simulink model "aurora_cpu_ch0_ver2_rtxsg"  (R2019b)
(part 3 of 4)

\"ch19\":{\"PauseBehavior\":\"0\",\"IdleBehavior\":\"0\",\"DefaultValueReg\":\"0\"},\"ch20\":{\"PauseBehavior\":\"0\",\"IdleBehavior\":\"0\",\"DefaultValueReg\":\"0\"},\"ch21\":{\"PauseBehavior\":\"0\",\"IdleBehavior\":\"0\",\"DefaultValueReg\":\"0\"},\"ch22\":{\"PauseBehavior\":\"0\",\"IdleBehavior\":\"0\",\"DefaultValueReg\":\"0\"},\"ch23\":{\"PauseBehavior\":\"0\",\"IdleBehavior\":\"0\",\"DefaultValueReg\":\"0\"},\"ch24\":{\"PauseBehavior\":\"0\",\"IdleBehavior\":\"0\",\"DefaultValueReg\":\"0\"},\"ch25\":{\"PauseBehavior\":\"0\",\"IdleBehavior\":\"0\",\"DefaultValueReg\":\"0\"},\"ch26\":{\"PauseBehavior\":\"0\",\"IdleBehavior\":\"0\",\"DefaultValueReg\":\"0\"},\"ch27\":{\"PauseBehavior\":\"0\",\"IdleBehavior\":\"0\",\"DefaultValueReg\":\"0\"},\"ch28\":{\"PauseBehavior\":\"0\",\"IdleBehavior\":\"0\",\"DefaultValueReg\":\"0\"},\"ch29\":{\"PauseBehavior\":\"0\",\"IdleBehavior\":\"0\",\"DefaultValueReg\":\"0\"},\"ch30\":{\"PauseBehavior\":\"0\",\"IdleBehavior\":\"0\",\"DefaultValueReg\":\"0\"},\"ch31\":{\"PauseBehavior\":\"0\",\"IdleBehavior\":\"0\",\"DefaultValueReg\":\"0\"}}}"  Expansion_DV_4B="{\"dv_Expansion_4B\":{\"ch0\":{\"PauseBehavior\":\"0\",\"IdleBehavior\":\"0\",\"DefaultValueReg\":\"0\"},\"ch1\":{\"PauseBehavior\":\"0\",\"IdleBehavior\":\"0\",\"DefaultValueReg\":\"0\"},\"ch2\":{\"PauseBehavior\":\"0\",\"IdleBehavior\":\"0\",\"DefaultValueReg\":\"0\"},\"ch3\":{\"PauseBehavior\":\"0\",\"IdleBehavior\":\"0\",\"DefaultValueReg\":\"0\"},\"ch4\":{\"PauseBehavior\":\"0\",\"IdleBehavior\":\"0\",\"DefaultValueReg\":\"0\"},\"ch5\":{\"PauseBehavior\":\"0\",\"IdleBehavior\":\"0\",\"DefaultValueReg\":\"0\"},\"ch6\":{\"PauseBehavior\":\"0\",\"IdleBehavior\":\"0\",\"DefaultValueReg\":\"0\"},\"ch7\":{\"PauseBehavior\":\"0\",\"IdleBehavior\":\"0\",\"DefaultValueReg\":\"0\"},\"ch8\":{\"PauseBehavior\":\"0\",\"IdleBehavior\":\"0\",\"DefaultValueReg\":\"0\"},\"ch9\":{\"PauseBehavior\":\"0\",\"IdleBehavior\":\"0\",\"DefaultValueReg\":\"0\"},\"ch10\":{\"PauseBehavior\":\"0\",\"IdleBehavior\":\"0\",\"DefaultValueReg\":\"0\"},\"ch11\":{\"PauseBehavior\":\"0\",\"IdleBehavior\":\"0\",\"DefaultValueReg\":\"0\"},\"ch12\":{\"PauseBehavior\":\"0\",\"IdleBehavior\":\"0\",\"DefaultValueReg\":\"0\"},\"ch13\":{\"PauseBehavior\":\"0\",\"IdleBehavior\":\"0\",\"DefaultValueReg\":\"0\"},\"ch14\":{\"PauseBehavior\":\"0\",\"IdleBehavior\":\"0\",\"DefaultValueReg\":\"0\"},\"ch15\":{\"PauseBehavior\":\"0\",\"IdleBehavior\":\"0\",\"DefaultValueReg\":\"0\"},\"ch16\":{\"PauseBehavior\":\"0\",\"IdleBehavior\":\"0\",\"DefaultValueReg\":\"0\"},\"ch17\":{\"PauseBehavior\":\"0\",\"IdleBehavior\":\"0\",\"DefaultValueReg\":\"0\"},\"ch18\":{\"PauseBehavior\":\"0\",\"IdleBehavior\":\"0\",\"DefaultValueReg\":\"0\"},\"ch19\":{\"PauseBehavior\":\"0\",\"IdleBehavior\":\"0\",\"DefaultValueReg\":\"0\"},\"ch20\":{\"PauseBehavior\":\"0\",\"IdleBehavior\":\"0\",\"DefaultValueReg\":\"0\"},\"ch21\":{\"PauseBehavior\":\"0\",\"IdleBehavior\":\"0\",\"DefaultValueReg\":\"0\"},\"ch22\":{\"PauseBehavior\":\"0\",\"IdleBehavior\":\"0\",\"DefaultValueReg\":\"0\"},\"ch23\":{\"PauseBehavior\":\"0\",\"IdleBehavior\":\"0\",\"DefaultValueReg\":\"0\"},\"ch24\":{\"PauseBehavior\":\"0\",\"IdleBehavior\":\"0\",\"DefaultValueReg\":\"0\"},\"ch25\":{\"PauseBehavior\":\"0\",\"IdleBehavior\":\"0\",\"DefaultValueReg\":\"0\"},\"ch26\":{\"PauseBehavior\":\"0\",\"IdleBehavior\":\"0\",\"DefaultValueReg\":\"0\"},\"ch27\":{\"PauseBehavior\":\"0\",\"IdleBehavior\":\"0\",\"DefaultValueReg\":\"0\"},\"ch28\":{\"PauseBehavior\":\"0\",\"IdleBehavior\":\"0\",\"DefaultValueReg\":\"0\"},\"ch29\":{\"PauseBehavior\":\"0\",\"IdleBehavior\":\"0\",\"DefaultValueReg\":\"0\"},\"ch30\":{\"PauseBehavior\":\"0\",\"IdleBehavior\":\"0\",\"DefaultValueReg\":\"0\"},\"ch31\":{\"PauseBehavior\":\"0\",\"IdleBehavior\":\"0\",\"DefaultValueReg\":\"0\"}}}"  Slot_DV_3A="{\"dv_3A\":{\"ch0\":{\"PauseBehavior\":\"0\",\"IdleBehavior\":\"0\",\"DefaultValueReg\":\"0\"},\"ch1\":{\"PauseBehavior\":\"0\",\"IdleBehavior\":\"0\",\"DefaultValueReg\":\"0\"},\"ch2\":{\"PauseBehavior\":\"0\",\"IdleBehavior\":\"0\",\"DefaultValueReg\":\"0\"},\"ch3\":{\"PauseBehavior\":\"0\",\"IdleBehavior\":\"0\",\"DefaultValueReg\":\"0\"},\"ch4\":{\"PauseBehavior\":\"0\",\"IdleBehavior\":\"0\",\"DefaultValueReg\":\"0\"},\"ch5\":{\"PauseBehavior\":\"0\",\"IdleBehavior\":\"0\",\"DefaultValueReg\":\"0\"},\"ch6\":{\"PauseBehavior\":\"0\",\"IdleBehavior\":\"0\",\"DefaultValueReg\":\"0\"},\"ch7\":{\"PauseBehavior\":\"0\",\"IdleBehavior\":\"0\",\"DefaultValueReg\":\"0\"},\"ch8\":{\"PauseBehavior\":\"0\",\"IdleBehavior\":\"0\",\"DefaultValueReg\":\"0\"},\"ch9\":{\"PauseBehavior\":\"0\",\"IdleBehavior\":\"0\",\"DefaultValueReg\":\"0\"},\"ch10\":{\"PauseBehavior\":\"0\",\"IdleBehavior\":\"0\",\"DefaultValueReg\":\"0\"},\"ch11\":{\"PauseBehavior\":\"0\",\"IdleBehavior\":\"0\",\"DefaultValueReg\":\"0\"},\"ch12\":{\"PauseBehavior\":\"0\",\"IdleBehavior\":\"0\",\"DefaultValueReg\":\"0\"},\"ch13\":{\"PauseBehavior\":\"0\",\"IdleBehavior\":\"0\",\"DefaultValueReg\":\"0\"},\"ch14\":{\"PauseBehavior\":\"0\",\"IdleBehavior\":\"0\",\"DefaultValueReg\":\"0\"},\"ch15\":{\"PauseBehavior\":\"0\",\"IdleBehavior\":\"0\",\"DefaultValueReg\":\"0\"},\"ch16\":{\"PauseBehavior\":\"0\",\"IdleBehavior\":\"0\",\"DefaultValueReg\":\"0\"},\"ch17\":{\"PauseBehavior\":\"0\",\"IdleBehavior\":\"0\",\"DefaultValueReg\":\"0\"},\"ch18\":{\"PauseBehavior\":\"0\",\"IdleBehavior\":\"0\",\"DefaultValueReg\":\"0\"},\"ch19\":{\"PauseBehavior\":\"0\",\"IdleBehavior\":\"0\",\"DefaultValueReg\":\"0\"},\"ch20\":{\"PauseBehavior\":\"0\",\"IdleBehavior\":\"0\",\"DefaultValueReg\":\"0\"},\"ch21\":{\"PauseBehavior\":\"0\",\"IdleBehavior\":\"0\",\"DefaultValueReg\":\"0\"},\"ch22\":{\"PauseBehavior\":\"0\",\"IdleBehavior\":\"0\",\"DefaultValueReg\":\"0\"},\"ch23\":{\"PauseBehavior\":\"0\",\"IdleBehavior\":\"0\",\"DefaultValueReg\":\"0\"},\"ch24\":{\"PauseBehavior\":\"0\",\"IdleBehavior\":\"0\",\"DefaultValueReg\":\"0\"},\"ch25\":{\"PauseBehavior\":\"0\",\"IdleBehavior\":\"0\",\"DefaultValueReg\":\"0\"},\"ch26\":{\"PauseBehavior\":\"0\",\"IdleBehavior\":\"0\",\"DefaultValueReg\":\"0\"},\"ch27\":{\"PauseBehavior\":\"0\",\"IdleBehavior\":\"0\",\"DefaultValueReg\":\"0\"},\"ch28\":{\"PauseBehavior\":\"0\",\"IdleBehavior\":\"0\",\"DefaultValueReg\":\"0\"},\"ch29\":{\"PauseBehavior\":\"0\",\"IdleBehavior\":\"0\",\"DefaultValueReg\":\"0\"},\"ch30\":{\"PauseBehavior\":\"0\",\"IdleBehavior\":\"0\",\"DefaultValueReg\":\"0\"},\"ch31\":{\"PauseBehavior\":\"0\",\"IdleBehavior\":\"0\",\"DefaultValueReg\":\"0\"}}}"  Slot_DV_3B="{\"dv_3B\":{\"ch0\":{\"PauseBehavior\":\"0\",\"IdleBehavior\":\"0\",\"DefaultValueReg\":\"0\"},\"ch1\":{\"PauseBehavior\":\"0\",\"IdleBehavior\":\"0\",\"DefaultValueReg\":\"0\"},\"ch2\":{\"PauseBehavior\":\"0\",\"IdleBehavior\":\"0\",\"DefaultValueReg\":\"0\"},\"ch3\":{\"PauseBehavior\":\"0\",\"IdleBehavior\":\"0\",\"DefaultValueReg\":\"0\"},\"ch4\":{\"PauseBehavior\":\"0\",\"IdleBehavior\":\"0\",\"DefaultValueReg\":\"0\"},\"ch5\":{\"PauseBehavior\":\"0\",\"IdleBehavior\":\"0\",\"DefaultValueReg\":\"0\"},\"ch6\":{\"PauseBehavior\":\"0\",\"IdleBehavior\":\"0\",\"DefaultValueReg\":\"0\"},\"ch7\":{\"PauseBehavior\":\"0\",\"IdleBehavior\":\"0\",\"DefaultValueReg\":\"0\"},\"ch8\":{\"PauseBehavior\":\"0\",\"IdleBehavior\":\"0\",\"DefaultValueReg\":\"0\"},\"ch9\":{\"PauseBehavior\":\"0\",\"IdleBehavior\":\"0\",\"DefaultValueReg\":\"0\"},\"ch10\":{\"PauseBehavior\":\"0\",\"IdleBehavior\":\"0\",\"DefaultValueReg\":\"0\"},\"ch11\":{\"PauseBehavior\":\"0\",\"IdleBehavior\":\"0\",\"DefaultValueReg\":\"0\"},\"ch12\":{\"PauseBehavior\":\"0\",\"IdleBehavior\":\"0\",\"DefaultValueReg\":\"0\"},\"ch13\":{\"PauseBehavior\":\"0\",\"IdleBehavior\":\"0\",\"DefaultValueReg\":\"0\"},\"ch14\":{\"PauseBehavior\":\"0\",\"IdleBehavior\":\"0\",\"DefaultValueReg\":\"0\"},\"ch15\":{\"PauseBehavior\":\"0\",\"IdleBehavior\":\"0\",\"DefaultValueReg\":\"0\"},\"ch16\":{\"PauseBehavior\":\"0\",\"IdleBehavior\":\"0\",\"DefaultValueReg\":\"0\"},\"ch17\":{\"PauseBehavior\":\"0\",\"IdleBehavior\":\"0\",\"DefaultValueReg\":\"0\"},\"ch18\":{\"PauseBehavior\":\"0\",\"IdleBehavior\":\"0\",\"DefaultValueReg\":\"0\"},\"ch19\":{\"PauseBehavior\":\"0\",\"IdleBehavior\":\"0\",\"DefaultValueReg\":\"0\"},\"ch20\":{\"PauseBehavior\":\"0\",\"IdleBehavior\":\"0\",\"DefaultValueReg\":\"0\"},\"ch21\":{\"PauseBehavior\":\"0\",\"IdleBehavior\":\"0\",\"DefaultValueReg\":\"0\"},\"ch22\":{\"PauseBehavior\":\"0\",\"IdleBehavior\":\"0\",\"DefaultValueReg\":\"0\"},\"ch23\":{\"PauseBehavior\":\"0\",\"IdleBehavior\":\"0\",\"DefaultValueReg\":\"0\"},\"ch24\":{\"PauseBehavior\":\"0\",\"IdleBehavior\":\"0\",\"DefaultValueReg\":\"0\"},\"ch25\":{\"PauseBehavior\":\"0\",\"IdleBehavior\":\"0\",\"DefaultValueReg\":\"0\"},\"ch26\":{\"PauseBehavior\":\"0\",\"IdleBehavior\":\"0\",\"DefaultValueReg\":\"0\"},\"ch27\":{\"PauseBehavior\":\"0\",\"IdleBehavior\":\"0\",\"DefaultValueReg\":\"0\"},\"ch28\":{\"PauseBehavior\":\"0\",\"IdleBehavior\":\"0\",\"DefaultValueReg\":\"0\"},\"ch29\":{\"PauseBehavior\":\"0\",\"IdleBehavior\":\"0\",\"DefaultValueReg\":\"0\"},\"ch30\":{\"PauseBehavior\":\"0\",\"IdleBehavior\":\"0\",\"DefaultValueReg\":\"0\"},\"ch31\":{\"PauseBehavior\":\"0\",\"IdleBehavior\":\"0\",\"DefaultValueReg\":\"0\"}}}"  Expansion_DV_3A="{\"dv_Expansion_3A\":{\"ch0\":{\"PauseBehavior\":\"0\",\"IdleBehavior\":\"0\",\"DefaultValueReg\":\"0\"},\"ch1\":{\"PauseBehavior\":\"0\",\"IdleBehavior\":\"0\",\"DefaultValueReg\":\"0\"},\"ch2\":{\"PauseBehavior\":\"0\",\"IdleBehavior\":\"0\",\"DefaultValueReg\":\"0\"},\"ch3\":{\"PauseBehavior\":\"0\",\"IdleBehavior\":\"0\",\"DefaultValueReg\":\"0\"},\"ch4\":{\"PauseBehavior\":\"0\",\"IdleBehavior\":\"0\",\"DefaultValueReg\":\"0\"},\"ch5\":{\"PauseBehavior\":\"0\",\"IdleBehavior\":\"0\",\"DefaultValueReg\":\"0\"},\"ch6\":{\"PauseBehavior\":\"0\",\"IdleBehavior\":\"0\",\"DefaultValueReg\":\"0\"},\"ch7\":{\"PauseBehavior\":\"0\",\"IdleBehavior\":\"0\",\"DefaultValueReg\":\"0\"},\"ch8\":{\"PauseBehavior\":\"0\",\"IdleBehavior\":\"0\",\"DefaultValueReg\":\"0\"},\"ch9\":{\"PauseBehavior\":\"0\",\"IdleBehavior\":\"0\",\"DefaultValueReg\":\"0\"},\"ch10\":{\"PauseBehavior\":\"0\",\"IdleBehavior\":\"0\",\"DefaultValueReg\":\"0\"},\"ch11\":{\"PauseBehavior\":\"0\",\"IdleBehavior\":\"0\",\"DefaultValueReg\":\"0\"},\"ch12\":{\"PauseBehavior\":\"0\",\"IdleBehavior\":\"0\",\"DefaultValueReg\":\"0\"},\"ch13\":{\"PauseBehavior\":\"0\",\"IdleBehavior\":\"0\",\"DefaultValueReg\":\"0\"},\"ch14\":{\"PauseBehavior\":\"0\",\"IdleBehavior\":\"0\",\"DefaultValueReg\":\"0\"},\"ch15\":{\"PauseBehavior\":\"0\",\"IdleBehavior\":\"0\",\"DefaultValueReg\":\"0\"},\"ch16\":{\"PauseBehavior\":\"0\",\"IdleBehavior\":\"0\",\"DefaultValueReg\":\"0\"},\"ch17\":{\"PauseBehavior\":\"0\",\"IdleBehavior\":\"0\",\"DefaultValueReg\":\"0\"},\"ch18\":{\"PauseBehavior\":\"0\",\"IdleBehavior\":\"0\",\"DefaultValueReg\":\"0\"},\"ch19\":{\"PauseBehavior\":\"0\",\"IdleBehavior\":\"0\",\"DefaultValueReg\":\"0\"},\"ch20\":{\"PauseBehavior\":\"0\",\"IdleBehavior\":\"0\",\"DefaultValueReg\":\"0\"},\"ch21\":{\"PauseBehavior\":\"0\",\"IdleBehavior\":\"0\",\"DefaultValueReg\":\"0\"},\"ch22\":{\"PauseBehavior\":\"0\",\"IdleBehavior\":\"0\",\"DefaultValueReg\":\"0\"},\"ch23\":{\"PauseBehavior\":\"0\",\"IdleBehavior\":\"0\",\"DefaultValueReg\":\"0\"},\"ch24\":{\"PauseBehavior\":\"0\",\"IdleBehavior\":\"0\",\"DefaultValueReg\":\"0\"},\"ch25\":{\"PauseBehavior\":\"0\",\"IdleBehavior\":\"0\",\"DefaultValueReg\":\"0\"},\"ch26\":{\"PauseBehavior\":\"0\",\"IdleBehavior\":\"0\",\"DefaultValueReg\":\"0\"},\"ch27\":{\"PauseBehavior\":\"0\",\"IdleBehavior\":\"0\",\"DefaultValueReg\":\"0\"},\"ch28\":{\"PauseBehavior\":\"0\",\"IdleBehavior\":\"0\",\"DefaultValueReg\":\"0\"},\"ch29\":{\"PauseBehavior\":\"0\",\"IdleBehavior\":\"0\",\"DefaultValueReg\":\"0\"},\"ch30\":{\"PauseBehavior\":\"0\",\"IdleBehavior\":\"0\",\"DefaultValueReg\":\"0\"},\"ch31\":{\"PauseBehavior\":\"0\",\"IdleBehavior\":\"0\",\"DefaultValueReg\":\"0\"}}}"  Expansion_DV_3B="{\"dv_Expansion_3B\":{\"ch0\":{\"PauseBehavior\":\"0\",\"IdleBehavior\":\"0\",\"DefaultValueReg\":\"0\"},\"ch1\":{\"PauseBehavior\":\"0\",\"IdleBehavior\":\"0\",\"DefaultValueReg\":\"0\"},\"ch2\":{\"PauseBehavior\":\"0\",\"IdleBehavior\":\"0\",\"DefaultValueReg\":\"0\"},\"ch3\":{\"PauseBehavior\":\"0\",\"IdleBehavior\":\"0\",\"DefaultValueReg\":\"0\"},\"ch4\":{\"PauseBehavior\":\"0\",\"IdleBehavior\":\"0\",\"DefaultValueReg\":\"0\"},\"ch5\":{\"PauseBehavior\":\"0\",\"IdleBehavior\":\"0\",\"DefaultValueReg\":\"0\"},\"ch6\":{\"PauseBehavior\":\"0\",\"IdleBehavior\":\"0\",\"DefaultValueReg\":\"0\"},\"ch7\":{\"PauseBehavior\":\"0\",\"IdleBehavior\":\"0\",\"DefaultValueReg\":\"0\"},\"ch8\":{\"PauseBehavior\":\"0\",\"IdleBehavior\":\"0\",\"DefaultValueReg\":\"0\"},\"ch9\":{\"PauseBehavior\":\"0\",\"IdleBehavior\":\"0\",\"DefaultValueReg\":\"0\"},\"ch10\":{\"PauseBehavior\":\"0\",\"IdleBehavior\":\"0\",\"DefaultValueReg\":\"0\"},\"ch11\":{\"PauseBehavior\":\"0\",\"IdleBehavior\":\"0\",\"DefaultValueReg\":\"0\"},\"ch12\":{\"PauseBehavior\":\"0\",\"IdleBehavior\":\"0\",\"DefaultValueReg\":\"0\"},\"ch13\":{\"PauseBehavior\":\"0\",\"IdleBehavior\":\"0\",\"DefaultValueReg\":\"0\"},\"ch14\":{\"PauseBehavior\":\"0\",\"IdleBehavior\":\"0\",\"DefaultValueReg\":\"0\"},\"ch15\":{\"PauseBehavior\":\"0\",\"IdleBehavior\":\"0\",\"DefaultValueReg\":\"0\"},\"ch16\":{\"PauseBehavior\":\"0\",\"IdleBehavior\":\"0\",\"DefaultValueReg\":\"0\"},\"ch17\":{\"PauseBehavior\":\"0\",\"IdleBehavior\":\"0\",\"DefaultValueReg\":\"0\"},\"ch18\":{\"PauseBehavior\":\"0\",\"IdleBehavior\":\"0\",\"DefaultValueReg\":\"0\"},\"ch19\":{\"PauseBehavior\":\"0\",\"IdleBehavior\":\"0\",\"DefaultValueReg\":\"0\"},\"ch20\":{\"PauseBehavior\":\"0\",\"IdleBehavior\":\"0\",\"DefaultValueReg\":\"0\"},\"ch21\":{\"PauseBehavior\":\"0\",\"IdleBehavior\":\"0\",\"DefaultValueReg\":\"0\"},\"ch22\":{\"PauseBehavior\":\"0\",\"IdleBehavior\":\"0\",\"DefaultValueReg\":\"0\"},\"ch23\":{\"PauseBehavior\":\"0\",\"IdleBehavior\":\"0\",\"DefaultValueReg\":\"0\"},\"ch24\":{\"PauseBehavior\":\"0\",\"IdleBehavior\":\"0\",\"DefaultValueReg\":\"0\"},\"ch25\":{\"PauseBehavior\":\"0\",\"IdleBehavior\":\"0\",\"DefaultValueReg\":\"0\"},\"ch26\":{\"PauseBehavior\":\"0\",\"IdleBehavior\":\"0\",\"DefaultValueReg\":\"0\"},\"ch27\":{\"PauseBehavior\":\"0\",\"IdleBehavior\":\"0\",\"DefaultValueReg\":\"0\"},\"ch28\":{\"PauseBehavior\":\"0\",\"IdleBehavior\":\"0\",\"DefaultValueReg\":\"0\"},\"ch29\":{\"PauseBehavior\":\"0\",\"IdleBehavior\":\"0\",\"DefaultValueReg\":\"0\"},\"ch30\":{\"PauseBehavior\":\"0\",\"IdleBehavior\":\"0\",\"DefaultValueReg\":\"0\"},\"ch31\":{\"PauseBehavior\":\"0\",\"IdleBehavior\":\"0\",\"DefaultValueReg\":\"0\"}}}"  Slot_DV_2A="{\"dv_2A\":{\"ch0\":{\"PauseBehavior\":\"0\",\"IdleBehavior\":\"0\",\"DefaultValueReg\":\"0\"},\"ch1\":{\"PauseBehavior\":\"0\",\"IdleBehavior\":\"0\",\"DefaultValueReg\":\"0\"},\"ch2\":{\"PauseBehavior\":\"0\",\"IdleBehavior\":\"0\",\"DefaultValueReg\":\"0\"},\"ch3\":{\"PauseBehavior\":\"0\",\"IdleBehavior\":\"0\",\"DefaultValueReg\":\"0\"},\"ch4\":{\"PauseBehavior\":\"0\",\"IdleBehavior\":\"0\",\"DefaultValueReg\":\"0\"},\"ch5\":{\"PauseBehavior\":\"0\",\"IdleBehavior\":\"0\",\"DefaultValueReg\":\"0\"},\"ch6\":{\"PauseBehavior\":\"0\",\"IdleBehavior\":\"0\",\"DefaultValueReg\":\"0\"},\"ch7\":{\"PauseBehavior\":\"0\",\"IdleBehavior\":\"0\",\"DefaultValueReg\":\"0\"},\"ch8\":{\"PauseBehavior\":\"0\",\"IdleBehavior\":\"0\",\"DefaultValueReg\":\"0\"},\"ch9\":{\"PauseBehavior\":\"0\",\"IdleBehavior\":\"0\",\"DefaultValueReg\":\"0\"},\"ch10\":{\"PauseBehavior\":\"0\",\"IdleBehavior\":\"0\",\"DefaultValueReg\":\"0\"},\"ch11\":{\"PauseBehavior\":\"0\",\"IdleBehavior\":\"0\",\"DefaultValueReg\":\"0\"},\"ch12\":{\"PauseBehavior\":\"0\",\"IdleBehavior\":\"0\",\"DefaultValueReg\":\"0\"},\"ch13\":{\"PauseBehavior\":\"0\",\"IdleBehavior\":\"0\",\"DefaultValueReg\":\"0\"},\"ch14\":{\"PauseBehavior\":\"0\",\"IdleBehavior\":\"0\",\"DefaultValueReg\":\"0\"},\"ch15\":{\"PauseBehavior\":\"0\",\"IdleBehavior\":\"0\",\"DefaultValueReg\":\"0\"},\"ch16\":{\"PauseBehavior\":\"0\",\"IdleBehavior\":\"0\",\"DefaultValueReg\":\"0\"},\"ch17\":{\"PauseBehavior\":\"0\",\"IdleBehavior\":\"0\",\"DefaultValueReg\":\"0\"},\"ch18\":{\"PauseBehavior\":\"0\",\"IdleBehavior\":\"0\",\"DefaultValueReg\":\"0\"},\"ch19\":{\"PauseBehavior\":\"0\",\"IdleBehavior\":\"0\",\"DefaultValueReg\":\"0\"},\"ch20\":{\"PauseBehavior\":\"0\",\"IdleBehavior\":\"0\",\"DefaultValueReg\":\"0\"},\"ch21\":{\"PauseBehavior\":\"0\",\"IdleBehavior\":\"0\",\"DefaultValueReg\":\"0\"},\"ch22\":{\"PauseBehavior\":\"0\",\"IdleBehavior\":\"0\",\"DefaultValueReg\":\"0\"},\"ch23\":{\"PauseBehavior\":\"0\",\"IdleBehavior\":\"0\",\"DefaultValueReg\":\"0\"},\"ch24\":{\"PauseBehavior\":\"0\",\"IdleBehavior\":\"0\",\"DefaultValueReg\":\"0\"},\"ch25\":{\"PauseBehavior\":\"0\",\"IdleBehavior\":\"0\",\"DefaultValueReg\":\"0\"},\"ch26\":{\"PauseBehavior\":\"0\",\"IdleBehavior\":\"0\",\"DefaultValueReg\":\"0\"},\"ch27\":{\"PauseBehavior\":\"0\",\"IdleBehavior\":\"0\",\"DefaultValueReg\":\"0\"},\"ch28\":{\"PauseBehavior\":\"0\",\"IdleBehavior\":\"0\",\"DefaultValueReg\":\"0\"},\"ch29\":{\"PauseBehavior\":\"0\",\"IdleBehavior\":\"0\",\"DefaultValueReg\":\"0\"},\"ch30\":{\"PauseBehavior\":\"0\",\"IdleBehavior\":\"0\",\"DefaultValueReg\":\"0\"},\"ch31\":{\"PauseBehavior\":\"0\",\"IdleBehavior\":\"0\",\"DefaultValueReg\":\"0\"}}}"  Slot_DV_2B="{\"dv_2B\":{\"ch0\":{\"PauseBehavior\":\"0\",\"IdleBehavior\":\"0\",\"DefaultValueReg\":\"0\"},\"ch1\":{\"PauseBehavior\":\"0\",\"IdleBehavior\":\"0\",\"DefaultValueReg\":\"0\"},\"ch2\":{\"PauseBehavior\":\"0\",\"IdleBehavior\":\"0\",\"DefaultValueReg\":\"0\"},\"ch3\":{\"PauseBehavior\":\"0\",\"IdleBehavior\":\"0\",\"DefaultValueReg\":\"0\"},\"ch4\":{\"PauseBehavior\":\"0\",\"IdleBehavior\":\"0\",\"DefaultValueReg\":\"0\"},\"ch5\":{\"PauseBehavior\":\"0\",\"IdleBehavior\":\"0\",\"DefaultValueReg\":\"0\"},\"ch6\":{\"PauseBehavior\":\"0\",\"IdleBehavior\":\"0\",\"DefaultValueReg\":\"0\"},\"ch7\":{\"PauseBehavior\":\"0\",\"IdleBehavior\":\"0\",\"DefaultValueReg\":\"0\"},\"ch8\":{\"PauseBehavior\":\"0\",\"IdleBehavior\":\"0\",\"DefaultValueReg\":\"0\"},\"ch9\":{\"PauseBehavior\":\"0\",\"IdleBehavior\":\"0\",\"DefaultValueReg\":\"0\"},\"ch10\":{\"PauseBehavior\":\"0\",\"IdleBehavior\":\"0\",\"DefaultValueReg\":\"0\"},\"ch11\":{\"PauseBehavior\":\"0\",\"IdleBehavior\":\"0\",\"DefaultValueReg\":\"0\"},\"ch12\":{\"PauseBehavior\":\"0\",\"IdleBehavior\":\"0\",\"DefaultValueReg\":\"0\"},\"ch13\":{\"PauseBehavior\":\"0\",\"IdleBehavior\":\"0\",\"DefaultValueReg\":\"0\"},\"ch14\":{\"PauseBehavior\":\"0\",\"IdleBehavior\":\"0\",\"DefaultValueReg\":\"0\"},\"ch15\":{\"PauseBehavior\":\"0\",\"IdleBehavior\":\"0\",\"DefaultValueReg\":\"0\"},\"ch16\":{\"PauseBehavior\":\"0\",\"IdleBehavior\":\"0\",\"DefaultValueReg\":\"0\"},\"ch17\":{\"PauseBehavior\":\"0\",\"IdleBehavior\":\"0\",\"DefaultValueReg\":\"0\"},\"ch18\":{\"PauseBehavior\":\"0\",\"IdleBehavior\":\"0\",\"DefaultValueReg\":\"0\"},\"ch19\":{\"PauseBehavior\":\"0\",\"IdleBehavior\":\"0\",\"DefaultValueReg\":\"0\"},\"ch20\":{\"PauseBehavior\":\"0\",\"IdleBehavior\":\"0\",\"DefaultValueReg\":\"0\"},\"ch21\":{\"PauseBehavior\":\"0\",\"IdleBehavior\":\"0\",\"DefaultValueReg\":\"0\"},\"ch22\":{\"PauseBehavior\":\"0\",\"IdleBehavior\":\"0\",\"DefaultValueReg\":\"0\"},\"ch23\":{\"PauseBehavior\":\"0\",\"IdleBehavior\":\"0\",\"DefaultValueReg\":\"0\"},\"ch24\":{\"PauseBehavior\":\"0\",\"IdleBehavior\":\"0\",\"DefaultValueReg\":\"0\"},\"ch25\":{\"PauseBehavior\":\"0\",\"IdleBehavior\":\"0\",\"DefaultValueReg\":\"0\"},\"ch26\":{\"PauseBehavior\":\"0\",\"IdleBehavior\":\"0\",\"DefaultValueReg\":\"0\"},\"ch27\":{\"PauseBehavior\":\"0\",\"IdleBehavior\":\"0\",\"DefaultValueReg\":\"0\"},\"ch28\":{\"PauseBehavior\":\"0\",\"IdleBehavior\":\"0\",\"DefaultValueReg\":\"0\"},\"ch29\":{\"PauseBehavior\":\"0\",\"IdleBehavior\":\"0\",\"DefaultValueReg\":\"0\"},\"ch30\":{\"PauseBehavior\":\"0\",\"IdleBehavior\":\"0\",\"DefaultValueReg\":\"0\"},\"ch31\":{\"PauseBehavior\":\"0\",\"IdleBehavior\":\"0\",\"DefaultValueReg\":\"0\"}}}"  Expansion_DV_2A="{\"dv_Expansion_2A\":{\"ch0\":{\"PauseBehavior\":\"0\",\"IdleBehavior\":\"0\",\"DefaultValueReg\":\"0\"},\"ch1\":{\"PauseBehavior\":\"0\",\"IdleBehavior\":\"0\",\"DefaultValueReg\":\"0\"},\"ch2\":{\"PauseBehavior\":\"0\",\"IdleBehavior\":\"0\",\"DefaultValueReg\":\"0\"},\"ch3\":{\"PauseBehavior\":\"0\",\"IdleBehavior\":\"0\",\"DefaultValueReg\":\"0\"},\"ch4\":{\"PauseBehavior\":\"0\",\"IdleBehavior\":\"0\",\"DefaultValueReg\":\"0\"},\"ch5\":{\"PauseBehavior\":\"0\",\"IdleBehavior\":\"0\",\"DefaultValueReg\":\"0\"},\"ch6\":{\"PauseBehavior\":\"0\",\"IdleBehavior\":\"0\",\"DefaultValueReg\":\"0\"},\"ch7\":{\"PauseBehavior\":\"0\",\"IdleBehavior\":\"0\",\"DefaultValueReg\":\"0\"},\"ch8\":{\"PauseBehavior\":\"0\",\"IdleBehavior\":\"0\",\"DefaultValueReg\":\"0\"},\"ch9\":{\"PauseBehavior\":\"0\",\"IdleBehavior\":\"0\",\"DefaultValueReg\":\"0\"},\"ch10\":{\"PauseBehavior\":\"0\",\"IdleBehavior\":\"0\",\"DefaultValueReg\":\"0\"},\"ch11\":{\"PauseBehavior\":\"0\",\"IdleBehavior\":\"0\",\"DefaultValueReg\":\"0\"},\"ch12\":{\"PauseBehavior\":\"0\",\"IdleBehavior\":\"0\",\"DefaultValueReg\":\"0\"},\"ch13\":{\"PauseBehavior\":\"0\",\"IdleBehavior\":\"0\",\"DefaultValueReg\":\"0\"},\"ch14\":{\"PauseBehavior\":\"0\",\"IdleBehavior\":\"0\",\"DefaultValueReg\":\"0\"},\"ch15\":{\"PauseBehavior\":\"0\",\"IdleBehavior\":\"0\",\"DefaultValueReg\":\"0\"},\"ch16\":{\"PauseBehavior\":\"0\",\"IdleBehavior\":\"0\",\"DefaultValueReg\":\"0\"},\"ch17\":{\"PauseBehavior\":\"0\",\"IdleBehavior\":\"0\",\"DefaultValueReg\":\"0\"},\"ch18\":{\"PauseBehavior\":\"0\",\"IdleBehavior\":\"0\",\"DefaultValueReg\":\"0\"},\"ch19\":{\"PauseBehavior\":\"0\",\"IdleBehavior\":\"0\",\"DefaultValueReg\":\"0\"},\"ch20\":{\"PauseBehavior\":\"0\",\"IdleBehavior\":\"0\",\"DefaultValueReg\":\"0\"},\"ch21\":{\"PauseBehavior\":\"0\",\"IdleBehavior\":\"0\",\"DefaultValueReg\":\"0\"},\"ch22\":{\"PauseBehavior\":\"0\",\"IdleBehavior\":\"0\",\"DefaultValueReg\":\"0\"},\"ch23\":{\"PauseBehavior\":\"0\",\"IdleBehavior\":\"0\",\"DefaultValueReg\":\"0\"},\"ch24\":{\"PauseBehavior\":\"0\",\"IdleBehavior\":\"0\",\"DefaultValueReg\":\"0\"},\"ch25\":{\"PauseBehavior\":\"0\",\"IdleBehavior\":\"0\",\"DefaultValueReg\":\"0\"},\"ch26\":{\"PauseBehavior\":\"0\",\"IdleBehavior\":\"0\",\"DefaultValueReg\":\"0\"},\"ch27\":{\"PauseBehavior\":\"0\",\"IdleBehavior\":\"0\",\"DefaultValueReg\":\"0\"},\"ch28\":{\"PauseBehavior\":\"0\",\"IdleBehavior\":\"0\",\"DefaultValueReg\":\"0\"},\"ch29\":{\"PauseBehavior\":\"0\",\"IdleBehavior\":\"0\",\"DefaultValueReg\":\"0\"},\"ch30\":{\"PauseBehavior\":\"0\",\"IdleBehavior\":\"0\",\"DefaultValueReg\":\"0\"},\"ch31\":{\"PauseBehavior\":\"0\",\"IdleBehavior\":\"0\",\"DefaultValueReg\":\"0\"}}}"  Expansion_DV_2B="{\"dv_Expansion_2B\":{\"ch0\":{\"PauseBehavior\":\"0\",\"IdleBehavior\":\"0\",\"DefaultValueReg\":\"0\"},\"ch1\":{\"PauseBehavior\":\"0\",\"IdleBehavior\":\"0\",\"DefaultValueReg\":\"0\"},\"ch2\":{\"PauseBehavior\":\"0\",\"IdleBehavior\":\"0\",\"DefaultValueReg\":\"0\"},\"ch3\":{\"PauseBehavior\":\"0\",\"IdleBehavior\":\"0\",\"DefaultValueReg\":\"0\"},\"ch4\":{\"PauseBehavior\":\"0\",\"IdleBehavior\":\"0\",\"DefaultValueReg\":\"0\"},\"ch5\":{\"PauseBehavior\":\"0\",\"IdleBehavior\":\"0\",\"DefaultValueReg\":\"0\"},\"ch6\":{\"PauseBehavior\":\"0\",\"IdleBehavior\":\"0\",\"DefaultValueReg\":\"0\"},\"ch7\":{\"PauseBehavior\":\"0\",\"IdleBehavior\":\"0\",\"DefaultValueReg\":\"0\"},\"ch8\":{\"PauseBehavior\":\"0\",\"IdleBehavior\":\"0\",\"DefaultValueReg\":\"0\"},\"ch9\":{\"PauseBehavior\":\"0\",\"IdleBehavior\":\"0\",\"DefaultValueReg\":\"0\"},\"ch10\":{\"PauseBehavior\":\"0\",\"IdleBehavior\":\"0\",\"DefaultValueReg\":\"0\"},\"ch11\":{\"PauseBehavior\":\"0\",\"IdleBehavior\":\"0\",\"DefaultValueReg\":\"0\"},\"ch12\":{\"PauseBehavior\":\"0\",\"IdleBehavior\":\"0\",\"DefaultValueReg\":\"0\"},\"ch13\":{\"PauseBehavior\":\"0\",\"IdleBehavior\":\"0\",\"DefaultValueReg\":\"0\"},\"ch14\":{\"PauseBehavior\":\"0\",\"IdleBehavior\":\"0\",\"DefaultValueReg\":\"0\"},\"ch15\":{\"PauseBehavior\":\"0\",\"IdleBehavior\":\"0\",\"DefaultValueReg\":\"0\"},\"ch16\":{\"PauseBehavior\":\"0\",\"IdleBehavior\":\"0\",\"DefaultValueReg\":\"0\"},\"ch17\":{\"PauseBehavior\":\"0\",\"IdleBehavior\":\"0\",\"DefaultValueReg\":\"0\"},\"ch18\":{\"PauseBehavior\":\"0\",\"IdleBehavior\":\"0\",\"DefaultValueReg\":\"0\"},\"ch19\":{\"PauseBehavior\":\"0\",\"IdleBehavior\":\"0\",\"DefaultValueReg\":\"0\"},\"ch20\":{\"PauseBehavior\":\"0\",\"IdleBehavior\":\"0\",\"DefaultValueReg\":\"0\"},\"ch21\":{\"PauseBehavior\":\"0\",\"IdleBehavior\":\"0\",\"DefaultValueReg\":\"0\"},\"ch22\":{\"PauseBehavior\":\"0\",\"IdleBehavior\":\"0\",\"DefaultValueReg\":\"0\"},\"ch23\":{\"PauseBehavior\":\"0\",\"IdleBehavior\":\"0\",\"DefaultValueReg\":\"0\"},\"ch24\":{\"PauseBehavior\":\"0\",\"IdleBehavior\":\"0\",\"DefaultValueReg\":\"0\"},\"ch25\":{\"PauseBehavior\":\"0\",\"IdleBehavior\":\"0\",\"DefaultValueReg\":\"0\"},\"ch26\":{\"PauseBehavior\":\"0\",\"IdleBehavior\":\"0\",\"DefaultValueReg\":\"0\"},\"ch27\":{\"PauseBehavior\":\"0\",\"IdleBehavior\":\"0\",\"DefaultValueReg\":\"0\"},\"ch28\":{\"PauseBehavior\":\"0\",\"IdleBehavior\":\"0\",\"DefaultValueReg\":\"0\"},\"ch29\":{\"PauseBehavior\":\"0\",\"IdleBehavior\":\"0\",\"DefaultValueReg\":\"0\"},\"ch30\":{\"PauseBehavior\":\"0\",\"IdleBehavior\":\"0\",\"DefaultValueReg\":\"0\"},\"ch31\":{\"PauseBehavior\":\"0\",\"IdleBehavior\":\"0\",\"DefaultValueReg\":\"0\"}}}"  Slot_DV_1A="{\"dv_1A\":{\"ch0\":{\"PauseBehavior\":\"0\",\"IdleBehavior\":\"0\",\"DefaultValueReg\":\"0\"},\"ch1\":{\"PauseBehavior\":\"0\",\"IdleBehavior\":\"0\",\"DefaultValueReg\":\"0\"},\"ch2\":{\"PauseBehavior\":\"0\",\"IdleBehavior\":\"0\",\"DefaultValueReg\":\"0\"},\"ch3\":{\"PauseBehavior\":\"0\",\"IdleBehavior\":\"0\",\"DefaultValueReg\":\"0\"},\"ch4\":{\"PauseBehavior\":\"0\",\"IdleBehavior\":\"0\",\"DefaultValueReg\":\"0\"},\"ch5\":{\"PauseBehavior\":\"0\",\"IdleBehavior\":\"0\",\"DefaultValueReg\":\"0\"},\"ch6\":{\"PauseBehavior\":\"0\",\"IdleBehavior\":\"0\",\"DefaultValueReg\":\"0\"},\"ch7\":{\"PauseBehavior\":\"0\",\"IdleBehavior\":\"0\",\"DefaultValueReg\":\"0\"},\"ch8\":{\"PauseBehavior\":\"0\",\"IdleBehavior\":\"0\",\"DefaultValueReg\":\"0\"},\"ch9\":{\"PauseBehavior\":\"0\",\"IdleBehavior\":\"0\",\"DefaultValueReg\":\"0\"},\"ch10\":{\"PauseBehavior\":\"0\",\"IdleBehavior\":\"0\",\"DefaultValueReg\":\"0\"},\"ch11\":{\"PauseBehavior\":\"0\",\"IdleBehavior\":\"0\",\"DefaultValueReg\":\"0\"},\"ch12\":{\"PauseBehavior\":\"0\",\"IdleBehavior\":\"0\",\"DefaultValueReg\":\"0\"},\"ch13\":{\"PauseBehavior\":\"0\",\"IdleBehavior\":\"0\",\"DefaultValueReg\":\"0\"},\"ch14\":{\"PauseBehavior\":\"0\",\"IdleBehavior\":\"0\",\"DefaultValueReg\":\"0\"},\"ch15\":{\"PauseBehavior\":\"0\",\"IdleBehavior\":\"0\",\"DefaultValueReg\":\"0\"},\"ch16\":{\"PauseBehavior\":\"0\",\"IdleBehavior\":\"0\",\"DefaultValueReg\":\"0\"},\"ch17\":{\"PauseBehavior\":\"0\",\"IdleBehavior\":\"0\",\"DefaultValueReg\":\"0\"},\"ch18\":{\"PauseBehavior\":\"0\",\"IdleBehavior\":\"0\",\"DefaultValueReg\":\"0\"},\"ch19\":{\"PauseBehavior\":\"0\",\"IdleBehavior\":\"0\",\"DefaultValueReg\":\"0\"},\"ch20\":{\"PauseBehavior\":\"0\",\"IdleBehavior\":\"0\",\"DefaultValueReg\":\"0\"},\"ch21\":{\"PauseBehavior\":\"0\",\"IdleBehavior\":\"0\",\"DefaultValueReg\":\"0\"},\"ch22\":{\"PauseBehavior\":\"0\",\"IdleBehavior\":\"0\",\"DefaultValueReg\":\"0\"},\"ch23\":{\"PauseBehavior\":\"0\",\"IdleBehavior\":\"0\",\"DefaultValueReg\":\"0\"},\"ch24\":{\"PauseBehavior\":\"0\",\"IdleBehavior\":\"0\",\"DefaultValueReg\":\"0\"},\"ch25\":{\"PauseBehavior\":\"0\",\"IdleBehavior\":\"0\",\"DefaultValueReg\":\"0\"},\"ch26\":{\"PauseBehavior\":\"0\",\"IdleBehavior\":\"0\",\"DefaultValueReg\":\"0\"},\"ch27\":{\"PauseBehavior\":\"0\",\"IdleBehavior\":\"0\",\"DefaultValueReg\":\"0\"},\"ch28\":{\"PauseBehavior\":\"0\",\"IdleBehavior\":\"0\",\"DefaultValueReg\":\"0\"},\"ch29\":{\"PauseBehavior\":\"0\",\"IdleBehavior\":\"0\",\"DefaultValueReg\":\"0\"},\"ch30\":{\"PauseBehavior\":\"0\",\"IdleBehavior\":\"0\",\"DefaultValueReg\":\"0\"},\"ch31\":{\"PauseBehavior\":\"0\",\"IdleBehavior\":\"0\",\"DefaultValueReg\":\"0\"}}}"  Slot_DV_1B="{\"dv_1B\":{\"ch0\":{\"PauseBehavior\":\"0\",\"IdleBehavior\":\"0\",\"DefaultValueReg\":\"0\"},\"ch1\":{\"PauseBehavior\":\"0\",\"IdleBehavior\":\"0\",\"DefaultValueReg\":\"0\"},\"ch2\":{\"PauseBehavior\":\"0\",\"IdleBehavior\":\"0\",\"DefaultValueReg\":\"0\"},\"ch3\":{\"PauseBehavior\":\"0\",\"IdleBehavior\":\"0\",\"DefaultValueReg\":\"0\"},\"ch4\":{\"PauseBehavior\":\"0\",\"IdleBehavior\":\"0\",\"DefaultValueReg\":\"0\"},\"ch5\":{\"PauseBehavior\":\"0\",\"IdleBehavior\":\"0\",\"DefaultValueReg\":\"0\"},\"ch6\":{\"PauseBehavior\":\"0\",\"IdleBehavior\":\"0\",\"DefaultValueReg\":\"0\"},\"ch7\":{\"PauseBehavior\":\"0\",\"IdleBehavior\":\"0\",\"DefaultValueReg\":\"0\"},\"ch8\":{\"PauseBehavior\":\"0\",\"IdleBehavior\":\"0\",\"DefaultValueReg\":\"0\"},\"ch9\":{\"PauseBehavior\":\"0\",\"IdleBehavior\":\"0\",\"DefaultValueReg\":\"0\"},\"ch10\":{\"PauseBehavior\":\"0\",\"IdleBehavior\":\"0\",\"DefaultValueReg\":\"0\"},\"ch11\":{\"PauseBehavior\":\"0\",\"IdleBehavior\":\"0\",\"DefaultValueReg\":\"0\"},\"ch12\":{\"PauseBehavior\":\"0\",\"IdleBehavior\":\"0\",\"DefaultValueReg\":\"0\"},\"ch13\":{\"PauseBehavior\":\"0\",\"IdleBehavior\":\"0\",\"DefaultValueReg\":\"0\"},\"ch14\":{\"PauseBehavior\":\"0\",\"IdleBehavior\":\"0\",\"DefaultValueReg\":\"0\"},\"ch15\":{\"PauseBehavior\":\"0\",\"IdleBehavior\":\"0\",\"DefaultValueReg\":\"0\"},\"ch16\":{\"PauseBehavior\":\"0\",\"IdleBehavior\":\"0\",\"DefaultValueReg\":\"0\"},\"ch17\":{\"PauseBehavior\":\"0\",\"IdleBehavior\":\"0\",\"DefaultValueReg\":\"0\"},\"ch18\":{\"PauseBehavior\":\"0\",\"IdleBehavior\":\"0\",\"DefaultValueReg\":\"0\"},\"ch19\":{\"PauseBehavior\":\"0\",\"IdleBehavior\":\"0\",\"DefaultValueReg\":\"0\"},\"ch20\":{\"PauseBehavior\":\"0\",\"IdleBehavior\":\"0\",\"DefaultValueReg\":\"0\"},\"ch21\":{\"PauseBehavior\":\"0\",\"IdleBehavior\":\"0\",\"DefaultValueReg\":\"0\"},\"ch22\":{\"PauseBehavior\":\"0\",\"IdleBehavior\":\"0\",\"DefaultValueReg\":\"0\"},\"ch23\":{\"PauseBehavior\":\"0\",\"IdleBehavior\":\"0\",\"DefaultValueReg\":\"0\"},\"ch24\":{\"PauseBehavior\":\"0\",\"IdleBehavior\":\"0\",\"DefaultValueReg\":\"0\"},\"ch25\":{\"PauseBehavior\":\"0\",\"IdleBehavior\":\"0\",\"DefaultValueReg\":\"0\"},\"ch26\":{\"PauseBehavior\":\"0\",\"IdleBehavior\":\"0\",\"DefaultValueReg\":\"0\"},\"ch27\":{\"PauseBehavior\":\"0\",\"IdleBehavior\":\"0\",\"DefaultValueReg\":\"0\"},\"ch28\":{\"PauseBehavior\":\"0\",\"IdleBehavior\":\"0\",\"DefaultValueReg\":\"0\"},\"ch29\":{\"PauseBehavior\":\"0\",\"IdleBehavior\":\"0\",\"DefaultValueReg\":\"0\"},\"ch30\":{\"PauseBehavior\":\"0\",\"IdleBehavior\":\"0\",\"DefaultValueReg\":\"0\"},\"ch31\":{\"PauseBehavior\":\"0\",\"IdleBehavior\":\"0\",\"DefaultValueReg\":\"0\"}}}"  Slot_DV_1C="{\"dv_1C\":{\"ch0\":{\"PauseBehavior\":\"0\",\"IdleBehavior\":\"0\",\"DefaultValueReg\":\"0\"},\"ch1\":{\"PauseBehavior\":\"0\",\"IdleBehavior\":\"0\",\"DefaultValueReg\":\"0\"},\"ch2\":{\"PauseBehavior\":\"0\",\"IdleBehavior\":\"0\",\"DefaultValueReg\":\"0\"},\"ch3\":{\"PauseBehavior\":\"0\",\"IdleBehavior\":\"0\",\"DefaultValueReg\":\"0\"},\"ch4\":{\"PauseBehavior\":\"0\",\"IdleBehavior\":\"0\",\"DefaultValueReg\":\"0\"},\"ch5\":{\"PauseBehavior\":\"0\",\"IdleBehavior\":\"0\",\"DefaultValueReg\":\"0\"},\"ch6\":{\"PauseBehavior\":\"0\",\"IdleBehavior\":\"0\",\"DefaultValueReg\":\"0\"},\"ch7\":{\"PauseBehavior\":\"0\",\"IdleBehavior\":\"0\",\"DefaultValueReg\":\"0\"},\"ch8\":{\"PauseBehavior\":\"0\",\"IdleBehavior\":\"0\",\"DefaultValueReg\":\"0\"},\"ch9\":{\"PauseBehavior\":\"0\",\"IdleBehavior\":\"0\",\"DefaultValueReg\":\"0\"},\"ch10\":{\"PauseBehavior\":\"0\",\"IdleBehavior\":\"0\",\"DefaultValueReg\":\"0\"},\"ch11\":{\"PauseBehavior\":\"0\",\"IdleBehavior\":\"0\",\"DefaultValueReg\":\"0\"},\"ch12\":{\"PauseBehavior\":\"0\",\"IdleBehavior\":\"0\",\"DefaultValueReg\":\"0\"},\"ch13\":{\"PauseBehavior\":\"0\",\"IdleBehavior\":\"0\",\"DefaultValueReg\":\"0\"},\"ch14\":{\"PauseBehavior\":\"0\",\"IdleBehavior\":\"0\",\"DefaultValueReg\":\"0\"},\"ch15\":{\"PauseBehavior\":\"0\",\"IdleBehavior\":\"0\",\"DefaultValueReg\":\"0\"},\"ch16\":{\"PauseBehavior\":\"0\",\"IdleBehavior\":\"0\",\"DefaultValueReg\":\"0\"},\"ch17\":{\"PauseBehavior\":\"0\",\"IdleBehavior\":\"0\",\"DefaultValueReg\":\"0\"},\"ch18\":{\"PauseBehavior\":\"0\",\"IdleBehavior\":\"0\",\"DefaultValueReg\":\"0\"},\"ch19\":{\"PauseBehavior\":\"0\",\"IdleBehavior\":\"0\",\"DefaultValueReg\":\"0\"},\"ch20\":{\"PauseBehavior\":\"0\",\"IdleBehavior\":\"0\",\"DefaultValueReg\":\"0\"},\"ch21\":{\"PauseBehavior\":\"0\",\"IdleBehavior\":\"0\",\"DefaultValueReg\":\"0\"},\"ch22\":{\"PauseBehavior\":\"0\",\"IdleBehavior\":\"0\",\"DefaultValueReg\":\"0\"},\"ch23\":{\"PauseBehavior\":\"0\",\"IdleBehavior\":\"0\",\"DefaultValueReg\":\"0\"},\"ch24\":{\"PauseBehavior\":\"0\",\"IdleBehavior\":\"0\",\"DefaultValueReg\":\"0\"},\"ch25\":{\"PauseBehavior\":\"0\",\"IdleBehavior\":\"0\",\"DefaultValueReg\":\"0\"},\"ch26\":{\"PauseBehavior\":\"0\",\"IdleBehavior\":\"0\",\"DefaultValueReg\":\"0\"},\"ch27\":{\"PauseBehavior\":\"0\",\"IdleBehavior\":\"0\",\"DefaultValueReg\":\"0\"},\"ch28\":{\"PauseBehavior\":\"0\",\"IdleBehavior\":\"0\",\"DefaultValueReg\":\"0\"},\"ch29\":{\"PauseBehavior\":\"0\",\"IdleBehavior\":\"0\",\"DefaultValueReg\":\"0\"},\"ch30\":{\"PauseBehavior\":\"0\",\"IdleBehavior\":\"0\",\"DefaultValueReg\":\"0\"},\"ch31\":{\"PauseBehavior\":\"0\",\"IdleBehavior\":\"0\",\"DefaultValueReg\":\"0\"}}}"  Slot_DV_1D="{\"dv_1D\":{\"ch0\":{\"PauseBehavior\":\"0\",\"IdleBehavior\":\"0\",\"DefaultValueReg\":\"0\"},\"ch1\":{\"PauseBehavior\":\"0\",\"IdleBehavior\":\"0\",\"DefaultValueReg\":\"0\"},\"ch2\":{\"PauseBehavior\":\"0\",\"IdleBehavior\":\"0\",\"DefaultValueReg\":\"0\"},\"ch3\":{\"PauseBehavior\":\"0\",\"IdleBehavior\":\"0\",\"DefaultValueReg\":\"0\"},\"ch4\":{\"PauseBehavior\":\"0\",\"IdleBehavior\":\"0\",\"DefaultValueReg\":\"0\"},\"ch5\":{\"PauseBehavior\":\"0\",\"IdleBehavior\":\"0\",\"DefaultValueReg\":\"0\"},\"ch6\":{\"PauseBehavior\":\"0\",\"IdleBehavior\":\"0\",\"DefaultValueReg\":\"0\"},\"ch7\":{\"PauseBehavior\":\"0\",\"IdleBehavior\":\"0\",\"DefaultValueReg\":\"0\"},\"ch8\":{\"PauseBehavior\":\"0\",\"IdleBehavior\":\"0\",\"DefaultValueReg\":\"0\"},\"ch9\":{\"PauseBehavior\":\"0\",\"IdleBehavior\":\"0\",\"DefaultValueReg\":\"0\"},\"ch10\":{\"PauseBehavior\":\"0\",\"IdleBehavior\":\"0\",\"DefaultValueReg\":\"0\"},\"ch11\":{\"PauseBehavior\":\"0\",\"IdleBehavior\":\"0\",\"DefaultValueReg\":\"0\"},\"ch12\":{\"PauseBehavior\":\"0\",\"IdleBehavior\":\"0\",\"DefaultValueReg\":\"0\"},\"ch13\":{\"PauseBehavior\":\"0\",\"IdleBehavior\":\"0\",\"DefaultValueReg\":\"0\"},\"ch14\":{\"PauseBehavior\":\"0\",\"IdleBehavior\":\"0\",\"DefaultValueReg\":\"0\"},\"ch15\":{\"PauseBehavior\":\"0\",\"IdleBehavior\":\"0\",\"DefaultValueReg\":\"0\"},\"ch16\":{\"PauseBehavior\":\"0\",\"IdleBehavior\":\"0\",\"DefaultValueReg\":\"0\"},\"ch17\":{\"PauseBehavior\":\"0\",\"IdleBehavior\":\"0\",\"DefaultValueReg\":\"0\"},\"ch18\":{\"PauseBehavior\":\"0\",\"IdleBehavior\":\"0\",\"DefaultValueReg\":\"0\"},\"ch19\":{\"PauseBehavior\":\"0\",\"IdleBehavior\":\"0\",\"DefaultValueReg\":\"0\"},\"ch20\":{\"PauseBehavior\":\"0\",\"IdleBehavior\":\"0\",\"DefaultValueReg\":\"0\"},\"ch21\":{\"PauseBehavior\":\"0\",\"IdleBehavior\":\"0\",\"DefaultValueReg\":\"0\"},\"ch22\":{\"PauseBehavior\":\"0\",\"IdleBehavior\":\"0\",\"DefaultValueReg\":\"0\"},\"ch23\":{\"PauseBehavior\":\"0\",\"IdleBehavior\":\"0\",\"DefaultValueReg\":\"0\"},\"ch24\":{\"PauseBehavior\":\"0\",\"IdleBehavior\":\"0\",\"DefaultValueReg\":\"0\"},\"ch25\":{\"PauseBehavior\":\"0\",\"IdleBehavior\":\"0\",\"DefaultValueReg\":\"0\"},\"ch26\":{\"PauseBehavior\":\"0\",\"IdleBehavior\":\"0\",\"DefaultValueReg\":\"0\"},\"ch27\":{\"PauseBehavior\":\"0\",\"IdleBehavior\":\"0\",\"DefaultValueReg\":\"0\"},\"ch28\":{\"PauseBehavior\":\"0\",\"IdleBehavior\":\"0\",\"DefaultValueReg\":\"0\"},\"ch29\":{\"PauseBehavior\":\"0\",\"IdleBehavior\":\"0\",\"DefaultValueReg\":\"0\"},\"ch30\":{\"PauseBehavior\":\"0\",\"IdleBehavior\":\"0\",\"DefaultValueReg\":\"0\"},\"ch31\":{\"PauseBehavior\":\"0\",\"IdleBehavior\":\"0\",\"DefaultValueReg\":\"0\"}}}"  Slot_DV_1E="{\"dv_1E\":{\"ch0\":{\"PauseBehavior\":\"0\",\"IdleBehavior\":\"0\",\"DefaultValueReg\":\"0\"},\"ch1\":{\"PauseBehavior\":\"0\",\"IdleBehavior\":\"0\",\"DefaultValueReg\":\"0\"},\"ch2\":{\"PauseBehavior\":\"0\",\"IdleBehavior\":\"0\",\"DefaultValueReg\":\"0\"},\"ch3\":{\"PauseBehavior\":\"0\",\"IdleBehavior\":\"0\",\"DefaultValueReg\":\"0\"},\"ch4\":{\"PauseBehavior\":\"0\",\"IdleBehavior\":\"0\",\"DefaultValueReg\":\"0\"},\"ch5\":{\"PauseBehavior\":\"0\",\"IdleBehavior\":\"0\",\"DefaultValueReg\":\"0\"},\"ch6\":{\"PauseBehavior\":\"0\",\"IdleBehavior\":\"0\",\"DefaultValueReg\":\"0\"},\"ch7\":{\"PauseBehavior\":\"0\",\"IdleBehavior\":\"0\",\"DefaultValueReg\":\"0\"},\"ch8\":{\"PauseBehavior\":\"0\",\"IdleBehavior\":\"0\",\"DefaultValueReg\":\"0\"},\"ch9\":{\"PauseBehavior\":\"0\",\"IdleBehavior\":\"0\",\"DefaultValueReg\":\"0\"},\"ch10\":{\"PauseBehavior\":\"0\",\"IdleBehavior\":\"0\",\"DefaultValueReg\":\"0\"},\"ch11\":{\"PauseBehavior\":\"0\",\"IdleBehavior\":\"0\",\"DefaultValueReg\":\"0\"},\"ch12\":{\"PauseBehavior\":\"0\",\"IdleBehavior\":\"0\",\"DefaultValueReg\":\"0\"},\"ch13\":{\"PauseBehavior\":\"0\",\"IdleBehavior\":\"0\",\"DefaultValueReg\":\"0\"},\"ch14\":{\"PauseBehavior\":\"0\",\"IdleBehavior\":\"0\",\"DefaultValueReg\":\"0\"},\"ch15\":{\"PauseBehavior\":\"0\",\"IdleBehavior\":\"0\",\"DefaultValueReg\":\"0\"},\"ch16\":{\"PauseBehavior\":\"0\",\"IdleBehavior\":\"0\",\"DefaultValueReg\":\"0\"},\"ch17\":{\"PauseBehavior\":\"0\",\"IdleBehavior\":\"0\",\"DefaultValueReg\":\"0\"},\"ch18\":{\"PauseBehavior\":\"0\",\"IdleBehavior\":\"0\",\"DefaultValueReg\":\"0\"},\"ch19\":{\"PauseBehavior\":\"0\",\"IdleBehavior\":\"0\",\"DefaultValueReg\":\"0\"},\"ch20\":{\"PauseBehavior\":\"0\",\"IdleBehavior\":\"0\",\"DefaultValueReg\":\"0\"},\"ch21\":{\"PauseBehavior\":\"0\",\"IdleBehavior\":\"0\",\"DefaultValueReg\":\"0\"},\"ch22\":{\"PauseBehavior\":\"0\",\"IdleBehavior\":\"0\",\"DefaultValueReg\":\"0\"},\"ch23\":{\"PauseBehavior\":\"0\",\"IdleBehavior\":\"0\",\"DefaultValueReg\":\"0\"},\"ch24\":{\"PauseBehavior\":\"0\",\"IdleBehavior\":\"0\",\"DefaultValueReg\":\"0\"},\"ch25\":{\"PauseBehavior\":\"0\",\"IdleBehavior\":\"0\",\"DefaultValueReg\":\"0\"},\"ch26\":{\"PauseBehavior\":\"0\",\"IdleBehavior\":\"0\",\"DefaultValueReg\":\"0\"},\"ch27\":{\"PauseBehavior\":\"0\",\"IdleBehavior\":\"0\",\"DefaultValueReg\":\"0\"},\"ch28\":{\"PauseBehavior\":\"0\",\"IdleBehavior\":\"0\",\"DefaultValueReg\":\"0\"},\"ch29\":{\"PauseBehavior\":\"0\",\"IdleBehavior\":\"0\",\"DefaultValueReg\":\"0\"},\"ch30\":{\"PauseBehavior\":\"0\",\"IdleBehavior\":\"0\",\"DefaultValueReg\":\"0\"},\"ch31\":{\"PauseBehavior\":\"0\",\"IdleBehavior\":\"0\",\"DefaultValueReg\":\"0\"}}}"  Slot_DV_1F="{\"dv_1F\":{\"ch0\":{\"PauseBehavior\":\"0\",\"IdleBehavior\":\"0\",\"DefaultValueReg\":\"0\"},\"ch1\":{\"PauseBehavior\":\"0\",\"IdleBehavior\":\"0\",\"DefaultValueReg\":\"0\"},\"ch2\":{\"PauseBehavior\":\"0\",\"IdleBehavior\":\"0\",\"DefaultValueReg\":\"0\"},\"ch3\":{\"PauseBehavior\":\"0\",\"IdleBehavior\":\"0\",\"DefaultValueReg\":\"0\"},\"ch4\":{\"PauseBehavior\":\"0\",\"IdleBehavior\":\"0\",\"DefaultValueReg\":\"0\"},\"ch5\":{\"PauseBehavior\":\"0\",\"IdleBehavior\":\"0\",\"DefaultValueReg\":\"0\"},\"ch6\":{\"PauseBehavior\":\"0\",\"IdleBehavior\":\"0\",\"DefaultValueReg\":\"0\"},\"ch7\":{\"PauseBehavior\":\"0\",\"IdleBehavior\":\"0\",\"DefaultValueReg\":\"0\"},\"ch8\":{\"PauseBehavior\":\"0\",\"IdleBehavior\":\"0\",\"DefaultValueReg\":\"0\"},\"ch9\":{\"PauseBehavior\":\"0\",\"IdleBehavior\":\"0\",\"DefaultValueReg\":\"0\"},\"ch10\":{\"PauseBehavior\":\"0\",\"IdleBehavior\":\"0\",\"DefaultValueReg\":\"0\"},\"ch11\":{\"PauseBehavior\":\"0\",\"IdleBehavior\":\"0\",\"DefaultValueReg\":\"0\"},\"ch12\":{\"PauseBehavior\":\"0\",\"IdleBehavior\":\"0\",\"DefaultValueReg\":\"0\"},\"ch13\":{\"PauseBehavior\":\"0\",\"IdleBehavior\":\"0\",\"DefaultValueReg\":\"0\"},\"ch14\":{\"PauseBehavior\":\"0\",\"IdleBehavior\":\"0\",\"DefaultValueReg\":\"0\"},\"ch15\":{\"PauseBehavior\":\"0\",\"IdleBehavior\":\"0\",\"DefaultValueReg\":\"0\"},\"ch16\":{\"PauseBehavior\":\"0\",\"IdleBehavior\":\"0\",\"DefaultValueReg\":\"0\"},\"ch17\":{\"PauseBehavior\":\"0\",\"IdleBehavior\":\"0\",\"DefaultValueReg\":\"0\"},\"ch18\":{\"PauseBehavior\":\"0\",\"IdleBehavior\":\"0\",\"DefaultValueReg\":\"0\"},\"ch19\":{\"PauseBehavior\":\"0\",\"IdleBehavior\":\"0\",\"DefaultValueReg\":\"0\"},\"ch20\":{\"PauseBehavior\":\"0\",\"IdleBehavior\":\"0\",\"DefaultValueReg\":\"0\"},\"ch21\":{\"PauseBehavior\":\"0\",\"IdleBehavior\":\"0\",\"DefaultValueReg\":\"0\"},\"ch22\":{\"PauseBehavior\":\"0\",\"IdleBehavior\":\"0\",\"DefaultValueReg\":\"0\"},\"ch23\":{\"PauseBehavior\":\"0\",\"IdleBehavior\":\"0\",\"DefaultValueReg\":\"0\"},\"ch24\":{\"PauseBehavior\":\"0\",\"IdleBehavior\":\"0\",\"DefaultValueReg\":\"0\"},\"ch25\":{\"PauseBehavior\":\"0\",\"IdleBehavior\":\"0\",\"DefaultValueReg\":\"0\"},\"ch26\":{\"PauseBehavior\":\"0\",\"IdleBehavior\":\"0\",\"DefaultValueReg\":\"0\"},\"ch27\":{\"PauseBehavior\":\"0\",\"IdleBehavior\":\"0\",\"DefaultValueReg\":\"0\"},\"ch28\":{\"PauseBehavior\":\"0\",\"IdleBehavior\":\"0\",\"DefaultValueReg\":\"0\"},\"ch29\":{\"PauseBehavior\":\"0\",\"IdleBehavior\":\"0\",\"DefaultValueReg\":\"0\"},\"ch30\":{\"PauseBehavior\":\"0\",\"IdleBehavior\":\"0\",\"DefaultValueReg\":\"0\"},\"ch31\":{\"PauseBehavior\":\"0\",\"IdleBehavior\":\"0\",\"DefaultValueReg\":\"0\"}}}"  Slot_DV_1G="{\"dv_1G\":{\"ch0\":{\"PauseBehavior\":\"0\",\"IdleBehavior\":\"0\",\"DefaultValueReg\":\"0\"},\"ch1\":{\"PauseBehavior\":\"0\",\"IdleBehavior\":\"0\",\"DefaultValueReg\":\"0\"},\"ch2\":{\"PauseBehavior\":\"0\",\"IdleBehavior\":\"0\",\"DefaultValueReg\":\"0\"},\"ch3\":{\"PauseBehavior\":\"0\",\"IdleBehavior\":\"0\",\"DefaultValueReg\":\"0\"},\"ch4\":{\"PauseBehavior\":\"0\",\"IdleBehavior\":\"0\",\"DefaultValueReg\":\"0\"},\"ch5\":{\"PauseBehavior\":\"0\",\"IdleBehavior\":\"0\",\"DefaultValueReg\":\"0\"},\"ch6\":{\"PauseBehavior\":\"0\",\"IdleBehavior\":\"0\",\"DefaultValueReg\":\"0\"},\"ch7\":{\"PauseBehavior\":\"0\",\"IdleBehavior\":\"0\",\"DefaultValueReg\":\"0\"},\"ch8\":{\"PauseBehavior\":\"0\",\"IdleBehavior\":\"0\",\"DefaultValueReg\":\"0\"},\"ch9\":{\"PauseBehavior\":\"0\",\"IdleBehavior\":\"0\",\"DefaultValueReg\":\"0\"},\"ch10\":{\"PauseBehavior\":\"0\",\"IdleBehavior\":\"0\",\"DefaultValueReg\":\"0\"},\"ch11\":{\"PauseBehavior\":\"0\",\"IdleBehavior\":\"0\",\"DefaultValueReg\":\"0\"},\"ch12\":{\"PauseBehavior\":\"0\",\"IdleBehavior\":\"0\",\"DefaultValueReg\":\"0\"},\"ch13\":{\"PauseBehavior\":\"0\",\"IdleBehavior\":\"0\",\"DefaultValueReg\":\"0\"},\"ch14\":{\"PauseBehavior\":\"0\",\"IdleBehavior\":\"0\",\"DefaultValueReg\":\"0\"},\"ch15\":{\"PauseBehavior\":\"0\",\"IdleBehavior\":\"0\",\"DefaultValueReg\":\"0\"},\"ch16\":{\"PauseBehavior\":\"0\",\"IdleBehavior\":\"0\",\"DefaultValueReg\":\"0\"},\"ch17\":{\"PauseBehavior\":\"0\",\"IdleBehavior\":\"0\",\"DefaultValueReg\":\"0\"},\"ch18\":{\"PauseBehavior\":\"0\",\"IdleBehavior\":\"0\",\"DefaultValueReg\":\"0\"},\"ch19\":{\"PauseBehavior\":\"0\",\"IdleBehavior\":\"0\",\"DefaultValueReg\":\"0\"},\"ch20\":{\"PauseBehavior\":\"0\",\"IdleBehavior\":\"0\",\"DefaultValueReg\":\"0\"},\"ch21\":{\"PauseBehavior\":\"0\",\"IdleBehavior\":\"0\",\"DefaultValueReg\":\"0\"},\"ch22\":{\"PauseBehavior\":\"0\",\"IdleBehavior\":\"0\",\"DefaultValueReg\":\"0\"},\"ch23\":{\"PauseBehavior\":\"0\",\"IdleBehavior\":\"0\",\"DefaultValueReg\":\"0\"},\"ch24\":{\"PauseBehavior\":\"0\",\"IdleBehavior\":\"0\",\"DefaultValueReg\":\"0\"},\"ch25\":{\"PauseBehavior\":\"0\",\"IdleBehavior\":\"0\",\"DefaultValueReg\":\"0\"},\"ch26\":{\"PauseBehavior\":\"0\",\"IdleBehavior\":\"0\",\"DefaultValueReg\":\"0\"},\"ch27\":{\"PauseBehavior\":\"0\",\"IdleBehavior\":\"0\",\"DefaultValueReg\":\"0\"},\"ch28\":{\"PauseBehavior\":\"0\",\"IdleBehavior\":\"0\",\"DefaultValueReg\":\"0\"},\"ch29\":{\"PauseBehavior\":\"0\",\"IdleBehavior\":\"0\",\"DefaultValueReg\":\"0\"},\"ch30\":{\"PauseBehavior\":\"0\",\"IdleBehavior\":\"0\",\"DefaultValueReg\":\"0\"},\"ch31\":{\"PauseBehavior\":\"0\",\"IdleBehavior\":\"0\",\"DefaultValueReg\":\"0\"}}}"  Slot_DV_1H="{\"dv_1H\":{\"ch0\":{\"PauseBehavior\":\"0\",\"IdleBehavior\":\"0\",\"DefaultValueReg\":\"0\"},\"ch1\":{\"PauseBehavior\":\"0\",\"IdleBehavior\":\"0\",\"DefaultValueReg\":\"0\"},\"ch2\":{\"PauseBehavior\":\"0\",\"IdleBehavior\":\"0\",\"DefaultValueReg\":\"0\"},\"ch3\":{\"PauseBehavior\":\"0\",\"IdleBehavior\":\"0\",\"DefaultValueReg\":\"0\"},\"ch4\":{\"PauseBehavior\":\"0\",\"IdleBehavior\":\"0\",\"DefaultValueReg\":\"0\"},\"ch5\":{\"PauseBehavior\":\"0\",\"IdleBehavior\":\"0\",\"DefaultValueReg\":\"0\"},\"ch6\":{\"PauseBehavior\":\"0\",\"IdleBehavior\":\"0\",\"DefaultValueReg\":\"0\"},\"ch7\":{\"PauseBehavior\":\"0\",\"IdleBehavior\":\"0\",\"DefaultValueReg\":\"0\"},\"ch8\":{\"PauseBehavior\":\"0\",\"IdleBehavior\":\"0\",\"DefaultValueReg\":\"0\"},\"ch9\":{\"PauseBehavior\":\"0\",\"IdleBehavior\":\"0\",\"DefaultValueReg\":\"0\"},\"ch10\":{\"PauseBehavior\":\"0\",\"IdleBehavior\":\"0\",\"DefaultValueReg\":\"0\"},\"ch11\":{\"PauseBehavior\":\"0\",\"IdleBehavior\":\"0\",\"DefaultValueReg\":\"0\"},\"ch12\":{\"PauseBehavior\":\"0\",\"IdleBehavior\":\"0\",\"DefaultValueReg\":\"0\"},\"ch13\":{\"PauseBehavior\":\"0\",\"IdleBehavior\":\"0\",\"DefaultValueReg\":\"0\"},\"ch14\":{\"PauseBehavior\":\"0\",\"IdleBehavior\":\"0\",\"DefaultValueReg\":\"0\"},\"ch15\":{\"PauseBehavior\":\"0\",\"IdleBehavior\":\"0\",\"DefaultValueReg\":\"0\"},\"ch16\":{\"PauseBehavior\":\"0\",\"IdleBehavior\":\"0\",\"DefaultValueReg\":\"0\"},\"ch17\":{\"PauseBehavior\":\"0\",\"IdleBehavior\":\"0\",\"DefaultValueReg\":\"0\"},\"ch18\":{\"PauseBehavior\":\"0\",\"IdleBehavior\":\"0\",\"DefaultValueReg\":\"0\"},\"ch19\":{\"PauseBehavior\":\"0\",\"IdleBehavior\":\"0\",\"DefaultValueReg\":\"0\"},\"ch20\":{\"PauseBehavior\":\"0\",\"IdleBehavior\":\"0\",\"DefaultValueReg\":\"0\"},\"ch21\":{\"PauseBehavior\":\"0\",\"IdleBehavior\":\"0\",\"DefaultValueReg\":\"0\"},\"ch22\":{\"PauseBehavior\":\"0\",\"IdleBehavior\":\"0\",\"DefaultValueReg\":\"0\"},\"ch23\":{\"PauseBehavior\":\"0\",\"IdleBehavior\":\"0\",\"DefaultValueReg\":\"0\"},\"ch24\":{\"PauseBehavior\":\"0\",\"IdleBehavior\":\"0\",\"DefaultValueReg\":\"0\"},\"ch25\":{\"PauseBehavior\":\"0\",\"IdleBehavior\":\"0\",\"DefaultValueReg\":\"0\"},\"ch26\":{\"PauseBehavior\":\"0\",\"IdleBehavior\":\"0\",\"DefaultValueReg\":\"0\"},\"ch27\":{\"PauseBehavior\":\"0\",\"IdleBehavior\":\"0\",\"DefaultValueReg\":\"0\"},\"ch28\":{\"PauseBehavior\":\"0\",\"IdleBehavior\":\"0\",\"DefaultValueReg\":\"0\"},\"ch29\":{\"PauseBehavior\":\"0\",\"IdleBehavior\":\"0\",\"DefaultValueReg\":\"0\"},\"ch30\":{\"PauseBehavior\":\"0\",\"IdleBehavior\":\"0\",\"DefaultValueReg\":\"0\"},\"ch31\":{\"PauseBehavior\":\"0\",\"IdleBehavior\":\"0\",\"DefaultValueReg\":\"0\"}}}"  Expansion_DV_1A="{\"dv_Expansion_1A\":{\"ch0\":{\"PauseBehavior\":\"0\",\"IdleBehavior\":\"0\",\"DefaultValueReg\":\"0\"},\"ch1\":{\"PauseBehavior\":\"0\",\"IdleBehavior\":\"0\",\"DefaultValueReg\":\"0\"},\"ch2\":{\"PauseBehavior\":\"0\",\"IdleBehavior\":\"0\",\"DefaultValueReg\":\"0\"},\"ch3\":{\"PauseBehavior\":\"0\",\"IdleBehavior\":\"0\",\"DefaultValueReg\":\"0\"},\"ch4\":{\"PauseBehavior\":\"0\",\"IdleBehavior\":\"0\",\"DefaultValueReg\":\"0\"},\"ch5\":{\"PauseBehavior\":\"0\",\"IdleBehavior\":\"0\",\"DefaultValueReg\":\"0\"},\"ch6\":{\"PauseBehavior\":\"0\",\"IdleBehavior\":\"0\",\"DefaultValueReg\":\"0\"},\"ch7\":{\"PauseBehavior\":\"0\",\"IdleBehavior\":\"0\",\"DefaultValueReg\":\"0\"},\"ch8\":{\"PauseBehavior\":\"0\",\"IdleBehavior\":\"0\",\"DefaultValueReg\":\"0\"},\"ch9\":{\"PauseBehavior\":\"0\",\"IdleBehavior\":\"0\",\"DefaultValueReg\":\"0\"},\"ch10\":{\"PauseBehavior\":\"0\",\"IdleBehavior\":\"0\",\"DefaultValueReg\":\"0\"},\"ch11\":{\"PauseBehavior\":\"0\",\"IdleBehavior\":\"0\",\"DefaultValueReg\":\"0\"},\"ch12\":{\"PauseBehavior\":\"0\",\"IdleBehavior\":\"0\",\"DefaultValueReg\":\"0\"},\"ch13\":{\"PauseBehavior\":\"0\",\"IdleBehavior\":\"0\",\"DefaultValueReg\":\"0\"},\"ch14\":{\"PauseBehavior\":\"0\",\"IdleBehavior\":\"0\",\"DefaultValueReg\":\"0\"},\"ch15\":{\"PauseBehavior\":\"0\",\"IdleBehavior\":\"0\",\"DefaultValueReg\":\"0\"},\"ch16\":{\"PauseBehavior\":\"0\",\"IdleBehavior\":\"0\",\"DefaultValueReg\":\"0\"},\"ch17\":{\"PauseBehavior\":\"0\",\"IdleBehavior\":\"0\",\"DefaultValueReg\":\"0\"},\"ch18\":{\"PauseBehavior\":\"0\",\"IdleBehavior\":\"0\",\"DefaultValueReg\":\"0\"},\"ch19\":{\"PauseBehavior\":\"0\",\"IdleBehavior\":\"0\",\"DefaultValueReg\":\"0\"},\"ch20\":{\"PauseBehavior\":\"0\",\"IdleBehavior\":\"0\",\"DefaultValueReg\":\"0\"},\"ch21\":{\"PauseBehavior\":\"0\",\"IdleBehavior\":\"0\",\"DefaultValueReg\":\"0\"},\"ch22\":{\"PauseBehavior\":\"0\",\"IdleBehavior\":\"0\",\"DefaultValueReg\":\"0\"},\"ch23\":{\"PauseBehavior\":\"0\",\"IdleBehavior\":\"0\",\"DefaultValueReg\":\"0\"},\"ch24\":{\"PauseBehavior\":\"0\",\"IdleBehavior\":\"0\",\"DefaultValueReg\":\"0\"},\"ch25\":{\"PauseBehavior\":\"0\",\"IdleBehavior\":\"0\",\"DefaultValueReg\":\"0\"},\"ch26\":{\"PauseBehavior\":\"0\",\"IdleBehavior\":\"0\",\"DefaultValueReg\":\"0\"},\"ch27\":{\"PauseBehavior\":\"0\",\"IdleBehavior\":\"0\",\"DefaultValueReg\":\"0\"},\"ch28\":{\"PauseBehavior\":\"0\",\"IdleBehavior\":\"0\",\"DefaultValueReg\":\"0\"},\"ch29\":{\"PauseBehavior\":\"0\",\"IdleBehavior\":\"0\",\"DefaultValueReg\":\"0\"},\"ch30\":{\"PauseBehavior\":\"0\",\"IdleBehavior\":\"0\",\"DefaultValueReg\":\"0\"},\"ch31\":{\"PauseBehavior\":\"0\",\"IdleBehavior\":\"0\",\"DefaultValueReg\":\"0\"}}}"  Expansion_DV_1B="{\"dv_Expansion_1B\":{\"ch0\":{\"PauseBehavior\":\"0\",\"IdleBehavior\":\"0\",\"DefaultValueReg\":\"0\"},\"ch1\":{\"PauseBehavior\":\"0\",\"IdleBehavior\":\"0\",\"DefaultValueReg\":\"0\"},\"ch2\":{\"PauseBehavior\":\"0\",\"IdleBehavior\":\"0\",\"DefaultValueReg\":\"0\"},\"ch3\":{\"PauseBehavior\":\"0\",\"IdleBehavior\":\"0\",\"DefaultValueReg\":\"0\"},\"ch4\":{\"PauseBehavior\":\"0\",\"IdleBehavior\":\"0\",\"DefaultValueReg\":\"0\"},\"ch5\":{\"PauseBehavior\":\"0\",\"IdleBehavior\":\"0\",\"DefaultValueReg\":\"0\"},\"ch6\":{\"PauseBehavior\":\"0\",\"IdleBehavior\":\"0\",\"DefaultValueReg\":\"0\"},\"ch7\":{\"PauseBehavior\":\"0\",\"IdleBehavior\":\"0\",\"DefaultValueReg\":\"0\"},\"ch8\":{\"PauseBehavior\":\"0\",\"IdleBehavior\":\"0\",\"DefaultValueReg\":\"0\"},\"ch9\":{\"PauseBehavior\":\"0\",\"IdleBehavior\":\"0\",\"DefaultValueReg\":\"0\"},\"ch10\":{\"PauseBehavior\":\"0\",\"IdleBehavior\":\"0\",\"DefaultValueReg\":\"0\"},\"ch11\":{\"PauseBehavior\":\"0\",\"IdleBehavior\":\"0\",\"DefaultValueReg\":\"0\"},\"ch12\":{\"PauseBehavior\":\"0\",\"IdleBehavior\":\"0\",\"DefaultValueReg\":\"0\"},\"ch13\":{\"PauseBehavior\":\"0\",\"IdleBehavior\":\"0\",\"DefaultValueReg\":\"0\"},\"ch14\":{\"PauseBehavior\":\"0\",\"IdleBehavior\":\"0\",\"DefaultValueReg\":\"0\"},\"ch15\":{\"PauseBehavior\":\"0\",\"IdleBehavior\":\"0\",\"DefaultValueReg\":\"0\"},\"ch16\":{\"PauseBehavior\":\"0\",\"IdleBehavior\":\"0\",\"DefaultValueReg\":\"0\"},\"ch17\":{\"PauseBehavior\":\"0\",\"IdleBehavior\":\"0\",\"DefaultValueReg\":\"0\"},\"ch18\":{\"PauseBehavior\":\"0\",\"IdleBehavior\":\"0\",\"DefaultValueReg\":\"0\"},\"ch19\":{\"PauseBehavior\":\"0\",\"IdleBehavior\":\"0\",\"DefaultValueReg\":\"0\"},\"ch20\":{\"PauseBehavior\":\"0\",\"IdleBehavior\":\"0\",\"DefaultValueReg\":\"0\"},\"ch21\":{\"PauseBehavior\":\"0\",\"IdleBehavior\":\"0\",\"DefaultValueReg\":\"0\"},\"ch22\":{\"PauseBehavior\":\"0\",\"IdleBehavior\":\"0\",\"DefaultValueReg\":\"0\"},\"ch23\":{\"PauseBehavior\":\"0\",\"IdleBehavior\":\"0\",\"DefaultValueReg\":\"0\"},\"ch24\":{\"PauseBehavior\":\"0\",\"IdleBehavior\":\"0\",\"DefaultValueReg\":\"0\"},\"ch25\":{\"PauseBehavior\":\"0\",\"IdleBehavior\":\"0\",\"DefaultValueReg\":\"0\"},\"ch26\":{\"PauseBehavior\":\"0\",\"IdleBehavior\":\"0\",\"DefaultValueReg\":\"0\"},\"ch27\":{\"PauseBehavior\":\"0\",\"IdleBehavior\":\"0\",\"DefaultValueReg\":\"0\"},\"ch28\":{\"PauseBehavior\":\"0\",\"IdleBehavior\":\"0\",\"DefaultValueReg\":\"0\"},\"ch29\":{\"PauseBehavior\":\"0\",\"IdleBehavior\":\"0\",\"DefaultValueReg\":\"0\"},\"ch30\":{\"PauseBehavior\":\"0\",\"IdleBehavior\":\"0\",\"DefaultValueReg\":\"0\"},\"ch31\":{\"PauseBehavior\":\"0\",\"IdleBehavior\":\"0\",\"DefaultValueReg\":\"0\"}}}"  Expansion_DV_1C="{\"dv_Expansion_1C\":{\"ch0\":{\"PauseBehavior\":\"0\",\"IdleBehavior\":\"0\",\"DefaultValueReg\":\"0\"},\"ch1\":{\"PauseBehavior\":\"0\",\"IdleBehavior\":\"0\",\"DefaultValueReg\":\"0\"},\"ch2\":{\"PauseBehavior\":\"0\",\"IdleBehavior\":\"0\",\"DefaultValueReg\":\"0\"},\"ch3\":{\"PauseBehavior\":\"0\",\"IdleBehavior\":\"0\",\"DefaultValueReg\":\"0\"},\"ch4\":{\"PauseBehavior\":\"0\",\"IdleBehavior\":\"0\",\"DefaultValueReg\":\"0\"},\"ch5\":{\"PauseBehavior\":\"0\",\"IdleBehavior\":\"0\",\"DefaultValueReg\":\"0\"},\"ch6\":{\"PauseBehavior\":\"0\",\"IdleBehavior\":\"0\",\"DefaultValueReg\":\"0\"},\"ch7\":{\"PauseBehavior\":\"0\",\"IdleBehavior\":\"0\",\"DefaultValueReg\":\"0\"},\"ch8\":{\"PauseBehavior\":\"0\",\"IdleBehavior\":\"0\",\"DefaultValueReg\":\"0\"},\"ch9\":{\"PauseBehavior\":\"0\",\"IdleBehavior\":\"0\",\"DefaultValueReg\":\"0\"},\"ch10\":{\"PauseBehavior\":\"0\",\"IdleBehavior\":\"0\",\"DefaultValueReg\":\"0\"},\"ch11\":{\"PauseBehavior\":\"0\",\"IdleBehavior\":\"0\",\"DefaultValueReg\":\"0\"},\"ch12\":{\"PauseBehavior\":\"0\",\"IdleBehavior\":\"0\",\"DefaultValueReg\":\"0\"},\"ch13\":{\"PauseBehavior\":\"0\",\"IdleBehavior\":\"0\",\"DefaultValueReg\":\"0\"},\"ch14\":{\"PauseBehavior\":\"0\",\"IdleBehavior\":\"0\",\"DefaultValueReg\":\"0\"},\"ch15\":{\"PauseBehavior\":\"0\",\"IdleBehavior\":\"0\",\"DefaultValueReg\":\"0\"},\"ch16\":{\"PauseBehavior\":\"0\",\"IdleBehavior\":\"0\",\"DefaultValueReg\":\"0\"},\"ch17\":{\"PauseBehavior\":\"0\",\"IdleBehavior\":\"0\",\"DefaultValueReg\":\"0\"},\"ch18\":{\"PauseBehavior\":\"0\",\"IdleBehavior\":\"0\",\"DefaultValueReg\":\"0\"},\"ch19\":{\"PauseBehavior\":\"0\",\"IdleBehavior\":\"0\",\"DefaultValueReg\":\"0\"},\"ch20\":{\"PauseBehavior\":\"0\",\"IdleBehavior\":\"0\",\"DefaultValueReg\":\"0\"},\"ch21\":{\"PauseBehavior\":\"0\",\"IdleBehavior\":\"0\",\"DefaultValueReg\":\"0\"},\"ch22\":{\"PauseBehavior\":\"0\",\"IdleBehavior\":\"0\",\"DefaultValueReg\":\"0\"},\"ch23\":{\"PauseBehavior\":\"0\",\"IdleBehavior\":\"0\",\"DefaultValueReg\":\"0\"},\"ch24\":{\"PauseBehavior\":\"0\",\"IdleBehavior\":\"0\",\"DefaultValueReg\":\"0\"},\"ch25\":{\"PauseBehavior\":\"0\",\"IdleBehavior\":\"0\",\"DefaultValueReg\":\"0\"},\"ch26\":{\"PauseBehavior\":\"0\",\"IdleBehavior\":\"0\",\"DefaultValueReg\":\"0\"},\"ch27\":{\"PauseBehavior\":\"0\",\"IdleBehavior\":\"0\",\"DefaultValueReg\":\"0\"},\"ch28\":{\"PauseBehavior\":\"0\",\"IdleBehavior\":\"0\",\"DefaultValueReg\":\"0\"},\"ch29\":{\"PauseBehavior\":\"0\",\"IdleBehavior\":\"0\",\"DefaultValueReg\":\"0\"},\"ch30\":{\"PauseBehavior\":\"0\",\"IdleBehavior\":\"0\",\"DefaultValueReg\":\"0\"},\"ch31\":{\"PauseBehavior\":\"0\",\"IdleBehavior\":\"0\",\"DefaultValueReg\":\"0\"}}}"  Expansion_DV_1D="{\"dv_Expansion_1D\":{\"ch0\":{\"PauseBehavior\":\"0\",\"IdleBehavior\":\"0\",\"DefaultValueReg\":\"0\"},\"ch1\":{\"PauseBehavior\":\"0\",\"IdleBehavior\":\"0\",\"DefaultValueReg\":\"0\"},\"ch2\":{\"PauseBehavior\":\"0\",\"IdleBehavior\":\"0\",\"DefaultValueReg\":\"0\"},\"ch3\":{\"PauseBehavior\":\"0\",\"IdleBehavior\":\"0\",\"DefaultValueReg\":\"0\"},\"ch4\":{\"PauseBehavior\":\"0\",\"IdleBehavior\":\"0\",\"DefaultValueReg\":\"0\"},\"ch5\":{\"PauseBehavior\":\"0\",\"IdleBehavior\":\"0\",\"DefaultValueReg\":\"0\"},\"ch6\":{\"PauseBehavior\":\"0\",\"IdleBehavior\":\"0\",\"DefaultValueReg\":\"0\"},\"ch7\":{\"PauseBehavior\":\"0\",\"IdleBehavior\":\"0\",\"DefaultValueReg\":\"0\"},\"ch8\":{\"PauseBehavior\":\"0\",\"IdleBehavior\":\"0\",\"DefaultValueReg\":\"0\"},\"ch9\":{\"PauseBehavior\":\"0\",\"IdleBehavior\":\"0\",\"DefaultValueReg\":\"0\"},\"ch10\":{\"PauseBehavior\":\"0\",\"IdleBehavior\":\"0\",\"DefaultValueReg\":\"0\"},\"ch11\":{\"PauseBehavior\":\"0\",\"IdleBehavior\":\"0\",\"DefaultValueReg\":\"0\"},\"ch12\":{\"PauseBehavior\":\"0\",\"IdleBehavior\":\"0\",\"DefaultValueReg\":\"0\"},\"ch13\":{\"PauseBehavior\":\"0\",\"IdleBehavior\":\"0\",\"DefaultValueReg\":\"0\"},\"ch14\":{\"PauseBehavior\":\"0\",\"IdleBehavior\":\"0\",\"DefaultValueReg\":\"0\"},\"ch15\":{\"PauseBehavior\":\"0\",\"IdleBehavior\":\"0\",\"DefaultValueReg\":\"0\"},\"ch16\":{\"PauseBehavior\":\"0\",\"IdleBehavior\":\"0\",\"DefaultValueReg\":\"0\"},\"ch17\":{\"PauseBehavior\":\"0\",\"IdleBehavior\":\"0\",\"DefaultValueReg\":\"0\"},\"ch18\":{\"PauseBehavior\":\"0\",\"IdleBehavior\":\"0\",\"DefaultValueReg\":\"0\"},\"ch19\":{\"PauseBehavior\":\"0\",\"IdleBehavior\":\"0\",\"DefaultValueReg\":\"0\"},\"ch20\":{\"PauseBehavior\":\"0\",\"IdleBehavior\":\"0\",\"DefaultValueReg\":\"0\"},\"ch21\":{\"PauseBehavior\":\"0\",\"IdleBehavior\":\"0\",\"DefaultValueReg\":\"0\"},\"ch22\":{\"PauseBehavior\":\"0\",\"IdleBehavior\":\"0\",\"DefaultValueReg\":\"0\"},\"ch23\":{\"PauseBehavior\":\"0\",\"IdleBehavior\":\"0\",\"DefaultValueReg\":\"0\"},\"ch24\":{\"PauseBehavior\":\"0\",\"IdleBehavior\":\"0\",\"DefaultValueReg\":\"0\"},\"ch25\":{\"PauseBehavior\":\"0\",\"IdleBehavior\":\"0\",\"DefaultValueReg\":\"0\"},\"ch26\":{\"PauseBehavior\":\"0\",\"IdleBehavior\":\"0\",\"DefaultValueReg\":\"0\"},\"ch27\":{\"PauseBehavior\":\"0\",\"IdleBehavior\":\"0\",\"DefaultValueReg\":\"0\"},\"ch28\":{\"PauseBehavior\":\"0\",\"IdleBehavior\":\"0\",\"DefaultValueReg\":\"0\"},\"ch29\":{\"PauseBehavior\":\"0\",\"IdleBehavior\":\"0\",\"DefaultValueReg\":\"0\"},\"ch30\":{\"PauseBehavior\":\"0\",\"IdleBehavior\":\"0\",\"DefaultValueReg\":\"0\"},\"ch31\":{\"PauseBehavior\":\"0\",\"IdleBehavior\":\"0\",\"DefaultValueReg\":\"0\"}}}"  Expansion_DV_1E="{\"dv_Expansion_1E\":{\"ch0\":{\"PauseBehavior\":\"0\",\"IdleBehavior\":\"0\",\"DefaultValueReg\":\"0\"},\"ch1\":{\"PauseBehavior\":\"0\",\"IdleBehavior\":\"0\",\"DefaultValueReg\":\"0\"},\"ch2\":{\"PauseBehavior\":\"0\",\"IdleBehavior\":\"0\",\"DefaultValueReg\":\"0\"},\"ch3\":{\"PauseBehavior\":\"0\",\"IdleBehavior\":\"0\",\"DefaultValueReg\":\"0\"},\"ch4\":{\"PauseBehavior\":\"0\",\"IdleBehavior\":\"0\",\"DefaultValueReg\":\"0\"},\"ch5\":{\"PauseBehavior\":\"0\",\"IdleBehavior\":\"0\",\"DefaultValueReg\":\"0\"},\"ch6\":{\"PauseBehavior\":\"0\",\"IdleBehavior\":\"0\",\"DefaultValueReg\":\"0\"},\"ch7\":{\"PauseBehavior\":\"0\",\"IdleBehavior\":\"0\",\"DefaultValueReg\":\"0\"},\"ch8\":{\"PauseBehavior\":\"0\",\"IdleBehavior\":\"0\",\"DefaultValueReg\":\"0\"},\"ch9\":{\"PauseBehavior\":\"0\",\"IdleBehavior\":\"0\",\"DefaultValueReg\":\"0\"},\"ch10\":{\"PauseBehavior\":\"0\",\"IdleBehavior\":\"0\",\"DefaultValueReg\":\"0\"},\"ch11\":{\"PauseBehavior\":\"0\",\"IdleBehavior\":\"0\",\"DefaultValueReg\":\"0\"},\"ch12\":{\"PauseBehavior\":\"0\",\"IdleBehavior\":\"0\",\"DefaultValueReg\":\"0\"},\"ch13\":{\"PauseBehavior\":\"0\",\"IdleBehavior\":\"0\",\"DefaultValueReg\":\"0\"},\"ch14\":{\"PauseBehavior\":\"0\",\"IdleBehavior\":\"0\",\"DefaultValueReg\":\"0\"},\"ch15\":{\"PauseBehavior\":\"0\",\"IdleBehavior\":\"0\",\"DefaultValueReg\":\"0\"},\"ch16\":{\"PauseBehavior\":\"0\",\"IdleBehavior\":\"0\",\"DefaultValueReg\":\"0\"},\"ch17\":{\"PauseBehavior\":\"0\",\"IdleBehavior\":\"0\",\"DefaultValueReg\":\"0\"},\"ch18\":{\"PauseBehavior\":\"0\",\"IdleBehavior\":\"0\",\"DefaultValueReg\":\"0\"},\"ch19\":{\"PauseBehavior\":\"0\",\"IdleBehavior\":\"0\",\"DefaultValueReg\":\"0\"},\"ch20\":{\"PauseBehavior\":\"0\",\"IdleBehavior\":\"0\",\"DefaultValueReg\":\"0\"},\"ch21\":{\"PauseBehavior\":\"0\",\"IdleBehavior\":\"0\",\"DefaultValueReg\":\"0\"},\"ch22\":{\"PauseBehavior\":\"0\",\"IdleBehavior\":\"0\",\"DefaultValueReg\":\"0\"},\"ch23\":{\"PauseBehavior\":\"0\",\"IdleBehavior\":\"0\",\"DefaultValueReg\":\"0\"},\"ch24\":{\"PauseBehavior\":\"0\",\"IdleBehavior\":\"0\",\"DefaultValueReg\":\"0\"},\"ch25\":{\"PauseBehavior\":\"0\",\"IdleBehavior\":\"0\",\"DefaultValueReg\":\"0\"},\"ch26\":{\"PauseBehavior\":\"0\",\"IdleBehavior\":\"0\",\"DefaultValueReg\":\"0\"},\"ch27\":{\"PauseBehavior\":\"0\",\"IdleBehavior\":\"0\",\"DefaultValueReg\":\"0\"},\"ch28\":{\"PauseBehavior\":\"0\",\"IdleBehavior\":\"0\",\"DefaultValueReg\":\"0\"},\"ch29\":{\"PauseBehavior\":\"0\",\"IdleBehavior\":\"0\",\"DefaultValueReg\":\"0\"},\"ch30\":{\"PauseBehavior\":\"0\",\"IdleBehavior\":\"0\",\"DefaultValueReg\":\"0\"},\"ch31\":{\"PauseBehavior\":\"0\",\"IdleBehavior\":\"0\",\"DefaultValueReg\":\"0\"}}}"  Expansion_DV_1F="{\"dv_Expansion_1F\":{\"ch0\":{\"PauseBehavior\":\"0\",\"IdleBehavior\":\"0\",\"DefaultValueReg\":\"0\"},\"ch1\":{\"PauseBehavior\":\"0\",\"IdleBehavior\":\"0\",\"DefaultValueReg\":\"0\"},\"ch2\":{\"PauseBehavior\":\"0\",\"IdleBehavior\":\"0\",\"DefaultValueReg\":\"0\"},\"ch3\":{\"PauseBehavior\":\"0\",\"IdleBehavior\":\"0\",\"DefaultValueReg\":\"0\"},\"ch4\":{\"PauseBehavior\":\"0\",\"IdleBehavior\":\"0\",\"DefaultValueReg\":\"0\"},\"ch5\":{\"PauseBehavior\":\"0\",\"IdleBehavior\":\"0\",\"DefaultValueReg\":\"0\"},\"ch6\":{\"PauseBehavior\":\"0\",\"IdleBehavior\":\"0\",\"DefaultValueReg\":\"0\"},\"ch7\":{\"PauseBehavior\":\"0\",\"IdleBehavior\":\"0\",\"DefaultValueReg\":\"0\"},\"ch8\":{\"PauseBehavior\":\"0\",\"IdleBehavior\":\"0\",\"DefaultValueReg\":\"0\"},\"ch9\":{\"PauseBehavior\":\"0\",\"IdleBehavior\":\"0\",\"DefaultValueReg\":\"0\"},\"ch10\":{\"PauseBehavior\":\"0\",\"IdleBehavior\":\"0\",\"DefaultValueReg\":\"0\"},\"ch11\":{\"PauseBehavior\":\"0\",\"IdleBehavior\":\"0\",\"DefaultValueReg\":\"0\"},\"ch12\":{\"PauseBehavior\":\"0\",\"IdleBehavior\":\"0\",\"DefaultValueReg\":\"0\"},\"ch13\":{\"PauseBehavior\":\"0\",\"IdleBehavior\":\"0\",\"DefaultValueReg\":\"0\"},\"ch14\":{\"PauseBehavior\":\"0\",\"IdleBehavior\":\"0\",\"DefaultValueReg\":\"0\"},\"ch15\":{\"PauseBehavior\":\"0\",\"IdleBehavior\":\"0\",\"DefaultValueReg\":\"0\"},\"ch16\":{\"PauseBehavior\":\"0\",\"IdleBehavior\":\"0\",\"DefaultValueReg\":\"0\"},\"ch17\":{\"PauseBehavior\":\"0\",\"IdleBehavior\":\"0\",\"DefaultValueReg\":\"0\"},\"ch18\":{\"PauseBehavior\":\"0\",\"IdleBehavior\":\"0\",\"DefaultValueReg\":\"0\"},\"ch19\":{\"PauseBehavior\":\"0\",\"IdleBehavior\":\"0\",\"DefaultValueReg\":\"0\"},\"ch20\":{\"PauseBehavior\":\"0\",\"IdleBehavior\":\"0\",\"DefaultValueReg\":\"0\"},\"ch21\":{\"PauseBehavior\":\"0\",\"IdleBehavior\":\"0\",\"DefaultValueReg\":\"0\"},\"ch22\":{\"PauseBehavior\":\"0\",\"IdleBehavior\":\"0\",\"DefaultValueReg\":\"0\"},\"ch23\":{\"PauseBehavior\":\"0\",\"IdleBehavior\":\"0\",\"DefaultValueReg\":\"0\"},\"ch24\":{\"PauseBehavior\":\"0\",\"IdleBehavior\":\"0\",\"DefaultValueReg\":\"0\"},\"ch25\":{\"PauseBehavior\":\"0\",\"IdleBehavior\":\"0\",\"DefaultValueReg\":\"0\"},\"ch26\":{\"PauseBehavior\":\"0\",\"IdleBehavior\":\"0\",\"DefaultValueReg\":\"0\"},\"ch27\":{\"PauseBehavior\":\"0\",\"IdleBehavior\":\"0\",\"DefaultValueReg\":\"0\"},\"ch28\":{\"PauseBehavior\":\"0\",\"IdleBehavior\":\"0\",\"DefaultValueReg\":\"0\"},\"ch29\":{\"PauseBehavior\":\"0\",\"IdleBehavior\":\"0\",\"DefaultValueReg\":\"0\"},\"ch30\":{\"PauseBehavior\":\"0\",\"IdleBehavior\":\"0\",\"DefaultValueReg\":\"0\"},\"ch31\":{\"PauseBehavior\":\"0\",\"IdleBehavior\":\"0\",\"DefaultValueReg\":\"0\"}}}"  Expansion_DV_1G="{\"dv_Expansion_1G\":{\"ch0\":{\"PauseBehavior\":\"0\",\"IdleBehavior\":\"0\",\"DefaultValueReg\":\"0\"},\"ch1\":{\"PauseBehavior\":\"0\",\"IdleBehavior\":\"0\",\"DefaultValueReg\":\"0\"},\"ch2\":{\"PauseBehavior\":\"0\",\"IdleBehavior\":\"0\",\"DefaultValueReg\":\"0\"},\"ch3\":{\"PauseBehavior\":\"0\",\"IdleBehavior\":\"0\",\"DefaultValueReg\":\"0\"},\"ch4\":{\"PauseBehavior\":\"0\",\"IdleBehavior\":\"0\",\"DefaultValueReg\":\"0\"},\"ch5\":{\"PauseBehavior\":\"0\",\"IdleBehavior\":\"0\",\"DefaultValueReg\":\"0\"},\"ch6\":{\"PauseBehavior\":\"0\",\"IdleBehavior\":\"0\",\"DefaultValueReg\":\"0\"},\"ch7\":{\"PauseBehavior\":\"0\",\"IdleBehavior\":\"0\",\"DefaultValueReg\":\"0\"},\"ch8\":{\"PauseBehavior\":\"0\",\"IdleBehavior\":\"0\",\"DefaultValueReg\":\"0\"},\"ch9\":{\"PauseBehavior\":\"0\",\"IdleBehavior\":\"0\",\"DefaultValueReg\":\"0\"},\"ch10\":{\"PauseBehavior\":\"0\",\"IdleBehavior\":\"0\",\"DefaultValueReg\":\"0\"},\"ch11\":{\"PauseBehavior\":\"0\",\"IdleBehavior\":\"0\",\"DefaultValueReg\":\"0\"},\"ch12\":{\"PauseBehavior\":\"0\",\"IdleBehavior\":\"0\",\"DefaultValueReg\":\"0\"},\"ch13\":{\"PauseBehavior\":\"0\",\"IdleBehavior\":\"0\",\"DefaultValueReg\":\"0\"},\"ch14\":{\"PauseBehavior\":\"0\",\"IdleBehavior\":\"0\",\"DefaultValueReg\":\"0\"},\"ch15\":{\"PauseBehavior\":\"0\",\"IdleBehavior\":\"0\",\"DefaultValueReg\":\"0\"},\"ch16\":{\"PauseBehavior\":\"0\",\"IdleBehavior\":\"0\",\"DefaultValueReg\":\"0\"},\"ch17\":{\"PauseBehavior\":\"0\",\"IdleBehavior\":\"0\",\"DefaultValueReg\":\"0\"},\"ch18\":{\"PauseBehavior\":\"0\",\"IdleBehavior\":\"0\",\"DefaultValueReg\":\"0\"},\"ch19\":{\"PauseBehavior\":\"0\",\"IdleBehavior\":\"0\",\"DefaultValueReg\":\"0\"},\"ch20\":{\"PauseBehavior\":\"0\",\"IdleBehavior\":\"0\",\"DefaultValueReg\":\"0\"},\"ch21\":{\"PauseBehavior\":\"0\",\"IdleBehavior\":\"0\",\"DefaultValueReg\":\"0\"},\"ch22\":{\"PauseBehavior\":\"0\",\"IdleBehavior\":\"0\",\"DefaultValueReg\":\"0\"},\"ch23\":{\"PauseBehavior\":\"0\",\"IdleBehavior\":\"0\",\"DefaultValueReg\":\"0\"},\"ch24\":{\"PauseBehavior\":\"0\",\"IdleBehavior\":\"0\",\"DefaultValueReg\":\"0\"},\"ch25\":{\"PauseBehavior\":\"0\",\"IdleBehavior\":\"0\",\"DefaultValueReg\":\"0\"},\"ch26\":{\"PauseBehavior\":\"0\",\"IdleBehavior\":\"0\",\"DefaultValueReg\":\"0\"},\"ch27\":{\"PauseBehavior\":\"0\",\"IdleBehavior\":\"0\",\"DefaultValueReg\":\"0\"},\"ch28\":{\"PauseBehavior\":\"0\",\"IdleBehavior\":\"0\",\"DefaultValueReg\":\"0\"},\"ch29\":{\"PauseBehavior\":\"0\",\"IdleBehavior\":\"0\",\"DefaultValueReg\":\"0\"},\"ch30\":{\"PauseBehavior\":\"0\",\"IdleBehavior\":\"0\",\"DefaultValueReg\":\"0\"},\"ch31\":{\"PauseBehavior\":\"0\",\"IdleBehavior\":\"0\",\"DefaultValueReg\":\"0\"}}}"  Expansion_DV_1H="{\"dv_Expansion_1H\":{\"ch0\":{\"PauseBehavior\":\"0\",\"IdleBehavior\":\"0\",\"DefaultValueReg\":\"0\"},\"ch1\":{\"PauseBehavior\":\"0\",\"IdleBehavior\":\"0\",\"DefaultValueReg\":\"0\"},\"ch2\":{\"PauseBehavior\":\"0\",\"IdleBehavior\":\"0\",\"DefaultValueReg\":\"0\"},\"ch3\":{\"PauseBehavior\":\"0\",\"IdleBehavior\":\"0\",\"DefaultValueReg\":\"0\"},\"ch4\":{\"PauseBehavior\":\"0\",\"IdleBehavior\":\"0\",\"DefaultValueReg\":\"0\"},\"ch5\":{\"PauseBehavior\":\"0\",\"IdleBehavior\":\"0\",\"DefaultValueReg\":\"0\"},\"ch6\":{\"PauseBehavior\":\"0\",\"IdleBehavior\":\"0\",\"DefaultValueReg\":\"0\"},\"ch7\":{\"PauseBehavior\":\"0\",\"IdleBehavior\":\"0\",\"DefaultValueReg\":\"0\"},\"ch8\":{\"PauseBehavior\":\"0\",\"IdleBehavior\":\"0\",\"DefaultValueReg\":\"0\"},\"ch9\":{\"PauseBehavior\":\"0\",\"IdleBehavior\":\"0\",\"DefaultValueReg\":\"0\"},\"ch10\":{\"PauseBehavior\":\"0\",\"IdleBehavior\":\"0\",\"DefaultValueReg\":\"0\"},\"ch11\":{\"PauseBehavior\":\"0\",\"IdleBehavior\":\"0\",\"DefaultValueReg\":\"0\"},\"ch12\":{\"PauseBehavior\":\"0\",\"IdleBehavior\":\"0\",\"DefaultValueReg\":\"0\"},\"ch13\":{\"PauseBehavior\":\"0\",\"IdleBehavior\":\"0\",\"DefaultValueReg\":\"0\"},\"ch14\":{\"PauseBehavior\":\"0\",\"IdleBehavior\":\"0\",\"DefaultValueReg\":\"0\"},\"ch15\":{\"PauseBehavior\":\"0\",\"IdleBehavior\":\"0\",\"DefaultValueReg\":\"0\"},\"ch16\":{\"PauseBehavior\":\"0\",\"IdleBehavior\":\"0\",\"DefaultValueReg\":\"0\"},\"ch17\":{\"PauseBehavior\":\"0\",\"IdleBehavior\":\"0\",\"DefaultValueReg\":\"0\"},\"ch18\":{\"PauseBehavior\":\"0\",\"IdleBehavior\":\"0\",\"DefaultValueReg\":\"0\"},\"ch19\":{\"PauseBehavior\":\"0\",\"IdleBehavior\":\"0\",\"DefaultValueReg\":\"0\"},\"ch20\":{\"PauseBehavior\":\"0\",\"IdleBehavior\":\"0\",\"DefaultValueReg\":\"0\"},\"ch21\":{\"PauseBehavior\":\"0\",\"IdleBehavior\":\"0\",\"DefaultValueReg\":\"0\"},\"ch22\":{\"PauseBehavior\":\"0\",\"IdleBehavior\":\"0\",\"DefaultValueReg\":\"0\"},\"ch23\":{\"PauseBehavior\":\"0\",\"IdleBehavior\":\"0\",\"DefaultValueReg\":\"0\"},\"ch24\":{\"PauseBehavior\":\"0\",\"IdleBehavior\":\"0\",\"DefaultValueReg\":\"0\"},\"ch25\":{\"PauseBehavior\":\"0\",\"IdleBehavior\":\"0\",\"DefaultValueReg\":\"0\"},\"ch26\":{\"PauseBehavior\":\"0\",\"IdleBehavior\":\"0\",\"DefaultValueReg\":\"0\"},\"ch27\":{\"PauseBehavior\":\"0\",\"IdleBehavior\":\"0\",\"DefaultValueReg\":\"0\"},\"ch28\":{\"PauseBehavior\":\"0\",\"IdleBehavior\":\"0\",\"DefaultValueReg\":\"0\"},\"ch29\":{\"PauseBehavior\":\"0\",\"IdleBehavior\":\"0\",\"DefaultValueReg\":\"0\"},\"ch30\":{\"PauseBehavior\":\"0\",\"IdleBehavior\":\"0\",\"DefaultValueReg\":\"0\"},\"ch31\":{\"PauseBehavior\":\"0\",\"IdleBehavior\":\"0\",\"DefaultValueReg\":\"0\"}}}"
      link override Version: version=hex2dec('24')  minorid=hex2dec('2')  CustomString=DUALSFP  Ts=1e-4  MaxFanoutMode=Auto
      settings: SourceProductName=RT-XSG
  Terminator : Terminator
  Terminator1 : Terminator
  Terminator2 : Terminator
  TimeStepSwitch : Subsystem
  TimestepGenerator : Subsystem
  Unpacking : Subsystem
  core0 : rtxsg_tools/core0  enabled=on  C_DATA_DEPTH=16384  C_EN_STRG_QUAL=on  C_ADV_TRIGGER=on  C_INPUT_PIPE_STAGES=0  ALL_PROBE_SAME_MU_CNT=2  probe0_gateways=i_nRst, i_ModelSync, iv_application_status, i_FPGASync
      settings: SourceProductName=RT-XSG
  data : rtxsg_tools/port0  enabled=on  core_enabled=on  core=core0  core_path=aurora_cpu_ch0_ver2_rtxsg/core0  probe_type=DATA_AND_TRIGGER
      settings: SourceProductName=RT-XSG
  fifo_Trig : rtxsg_tools/port0  enabled=on  core_enabled=on  core=core0  core_path=aurora_cpu_ch0_ver2_rtxsg/core0  probe_type=DATA_AND_TRIGGER
      settings: SourceProductName=RT-XSG
  fifo_tdata : rtxsg_tools/port0  enabled=on  core_enabled=on  core=core0  core_path=aurora_cpu_ch0_ver2_rtxsg/core0  probe_type=DATA_AND_TRIGGER
      settings: SourceProductName=RT-XSG
  fifo_tlast : rtxsg_tools/port0  enabled=on  core_enabled=on  core=core0  core_path=aurora_cpu_ch0_ver2_rtxsg/core0  probe_type=DATA_AND_TRIGGER
      settings: SourceProductName=RT-XSG
  fifo_tvalid : rtxsg_tools/port0  enabled=on  core_enabled=on  core=core0  core_path=aurora_cpu_ch0_ver2_rtxsg/core0  probe_type=DATA_AND_TRIGGER
      settings: SourceProductName=RT-XSG
  input_tdata : rtxsg_tools/port0  enabled=on  core_enabled=on  core=core0  core_path=aurora_cpu_ch0_ver2_rtxsg/core0  probe_type=DATA_AND_TRIGGER
      settings: SourceProductName=RT-XSG
  input_tlast : rtxsg_tools/port0  enabled=on  core_enabled=on  core=core0  core_path=aurora_cpu_ch0_ver2_rtxsg/core0  probe_type=DATA_AND_TRIGGER
      settings: SourceProductName=RT-XSG
  "input_tvalid " : rtxsg_tools/port0  enabled=on  core_enabled=on  core=core0  core_path=aurora_cpu_ch0_ver2_rtxsg/core0  probe_type=DATA_AND_TRIGGER
      settings: SourceProductName=RT-XSG
  last : rtxsg_tools/port0  enabled=on  core_enabled=on  core=core0  core_path=aurora_cpu_ch0_ver2_rtxsg/core0  probe_type=DATA_AND_TRIGGER
      settings: SourceProductName=RT-XSG
  out_data : rtxsg_tools/port0  enabled=on  core_enabled=on  core=core0  core_path=aurora_cpu_ch0_ver2_rtxsg/core0  probe_type=DATA_AND_TRIGGER
      settings: SourceProductName=RT-XSG
  post_tdata : rtxsg_tools/port0  enabled=on  core_enabled=on  core=core0  core_path=aurora_cpu_ch0_ver2_rtxsg/core0  probe_type=DATA_AND_TRIGGER
      settings: SourceProductName=RT-XSG
  post_tlast : rtxsg_tools/port0  enabled=on  core_enabled=on  core=core0  core_path=aurora_cpu_ch0_ver2_rtxsg/core0  probe_type=DATA_AND_TRIGGER
      settings: SourceProductName=RT-XSG
  post_tvalid : rtxsg_tools/port0  enabled=on  core_enabled=on  core=core0  core_path=aurora_cpu_ch0_ver2_rtxsg/core0  probe_type=DATA_AND_TRIGGER
      settings: SourceProductName=RT-XSG
  pre_tdata : rtxsg_tools/port0  enabled=on  core_enabled=on  core=core0  core_path=aurora_cpu_ch0_ver2_rtxsg/core0  probe_type=DATA_AND_TRIGGER
      settings: SourceProductName=RT-XSG
  pre_tlast : rtxsg_tools/port0  enabled=on  core_enabled=on  core=core0  core_path=aurora_cpu_ch0_ver2_rtxsg/core0  probe_type=DATA_AND_TRIGGER
      settings: SourceProductName=RT-XSG
  pre_tready : rtxsg_tools/port0  enabled=on  core_enabled=on  core=core0  core_path=aurora_cpu_ch0_ver2_rtxsg/core0  probe_type=DATA_AND_TRIGGER
      settings: SourceProductName=RT-XSG
  pre_tvalid : rtxsg_tools/port0  enabled=on  core_enabled=on  core=core0  core_path=aurora_cpu_ch0_ver2_rtxsg/core0  probe_type=DATA_AND_TRIGGER
      settings: SourceProductName=RT-XSG
  ready : rtxsg_tools/port0  enabled=on  core_enabled=on  core=core0  core_path=aurora_cpu_ch0_ver2_rtxsg/core0  probe_type=DATA_AND_TRIGGER
      settings: SourceProductName=RT-XSG
  userTStep : rtxsg_tools/port0  enabled=on  core_enabled=on  core=core0  core_path=aurora_cpu_ch0_ver2_rtxsg/core0  probe_type=DATA_AND_TRIGGER
      settings: SourceProductName=RT-XSG
  valid : rtxsg_tools/port0  enabled=on  core_enabled=on  core=core0  core_path=aurora_cpu_ch0_ver2_rtxsg/core0  probe_type=DATA_AND_TRIGGER
      settings: SourceProductName=RT-XSG
  wires:
  DataOUT/1 -> Terminator/1
  Constant/1 -> DataIN1/1
  StatusPacker/2(DataSync) -> DataOUT/3
  StatusPacker/1(DataOut) -> DataOUT/2
  Concat1/1 -> StatusPacker/1(Status)
  GenericHighSpeedComm_Aurora_8B10B_7Series/1 -> Assert3/1
  Inverter/1 -> Convert5/1
  Simulation State/3 -> Inverter/1
  GenericHighSpeedComm_Aurora_8B10B_7Series/14 -> Concat1/5
  GenericHighSpeedComm_Aurora_8B10B_7Series/13 -> Concat1/4
  GenericHighSpeedComm_Aurora_8B10B_7Series/12 -> Concat1/3
  GenericHighSpeedComm_Aurora_8B10B_7Series/11 -> Concat1/2
  Concat/1 -> Concat1/1  "Errors"
  GenericHighSpeedComm_Aurora_8B10B_7Series/3 -> Assert1/1
  GenericHighSpeedComm_Aurora_8B10B_7Series/4 -> Assert2/1
  GenericHighSpeedComm_Aurora_8B10B_7Series/5 -> Concat/1
  GenericHighSpeedComm_Aurora_8B10B_7Series/6 -> Concat/2
  GenericHighSpeedComm_Aurora_8B10B_7Series/7 -> Concat/3
  GenericHighSpeedComm_Aurora_8B10B_7Series/8 -> Concat/4
  GenericHighSpeedComm_Aurora_8B10B_7Series/9 -> Concat/5
  GenericHighSpeedComm_Aurora_8B10B_7Series/10 -> Concat/6
  GenericHighSpeedComm_Aurora_8B10B_7Series/2 -> Assert/1
  Assert3/1 -> Convert3/1  "Ready"
  LoadIN/1 -> Unpacking/1(LoadIn)
  LoadIN/2 -> Unpacking/2(LoadSof)
  Constant1/1 -> LoadIN/1
  Assert/1 -> Convert8/1, BitBasher/2, valid/1  "Valid"
  BitBasher/1 -> DataOUT/1, out_data/1
  Rate transition1/3 -> Delay3/1
  Assert2/1 -> Register1/1, BitBasher/1, data/1  "DataIn"
  Convert1/1 -> TimeStepSwitch/1(MasterTimeStep), Register1/2, Delay1/1, SOF_detector/2(last), last/1
  Constant5/1 -> Synchronization/2(SyncMode)
  Constant6/1 -> Synchronization/3(Delay)
  Unpacking/2(Delay) -> Terminator2/1
  Unpacking/1(SyncMode) -> Terminator1/1
  Convert3/1 -> ready/1, Rate transition1/4
  Convert7/1 -> pre_tready/1, AXI FIFO1/2
  SofToAxi1/4(reset) -> AXI FIFO1/1
  SofToAxi1/2(Valid) -> pre_tvalid/1, AXI FIFO1/3
  DataIN1/3 -> SofToAxi1/1(DataIn)
  SofToAxi1/1(Data) -> pre_tdata/1, AXI FIFO1/4
  AXI FIFO1/1 -> post_tvalid/1, GenericHighSpeedComm_Aurora_8B10B_7Series1/1
  DataIN1/4 -> SofToAxi1/2(SofIn)
  SofToAxi1/3(Last) -> pre_tlast/1, AXI FIFO1/5
  Assert5/1 -> Rate transition/3  "Last"
  Assert7/1 -> Convert7/1  "Ready"
  AXI FIFO1/3 -> GenericHighSpeedComm_Aurora_8B10B_7Series1/3, post_tlast/1
  Convert5/1 -> GenericHighSpeedComm_Aurora_8B10B_7Series1/4, GenericHighSpeedComm_Aurora_8B10B_7Series/4
  GenericHighSpeedComm_Aurora_8B10B_7Series1/5 -> Concat2/1
  GenericHighSpeedComm_Aurora_8B10B_7Series1/7 -> Concat2/3
  GenericHighSpeedComm_Aurora_8B10B_7Series1/3 -> Assert5/1
  GenericHighSpeedComm_Aurora_8B10B_7Series1/1 -> Assert7/1
  GenericHighSpeedComm_Aurora_8B10B_7Series1/4 -> Assert6/1
  GenericHighSpeedComm_Aurora_8B10B_7Series1/2 -> Assert4/1
  GenericHighSpeedComm_Aurora_8B10B_7Series1/9 -> Concat2/5
  GenericHighSpeedComm_Aurora_8B10B_7Series1/10 -> Concat2/6
  GenericHighSpeedComm_Aurora_8B10B_7Series1/14 -> Concat3/5
  GenericHighSpeedComm_Aurora_8B10B_7Series1/13 -> Concat3/4
  GenericHighSpeedComm_Aurora_8B10B_7Series1/8 -> Concat2/4
  GenericHighSpeedComm_Aurora_8B10B_7Series1/11 -> Concat3/2
  GenericHighSpeedComm_Aurora_8B10B_7Series1/12 -> Concat3/3
  Concat2/1 -> Concat3/1  "Errors"
  GenericHighSpeedComm_Aurora_8B10B_7Series1/6 -> Concat2/2
  Assert4/1 -> Rate transition/2  "Valid"
  Assert6/1 -> Rate transition/1  "DataIn"
  Rate transition/2 -> BitBasher1/2
  Rate transition/1 -> BitBasher1/1
  Constant7/1 -> Rate transition/4
  Concat3/1 -> StatusPacker1/1(Status)
  StatusPacker1/1(DataOut) -> DataOUT/5
  StatusPacker1/2(DataSync) -> DataOUT/6
  BitBasher1/1 -> DataOUT/4
  AXI FIFO1/2 -> post_tdata/1, GenericHighSpeedComm_Aurora_8B10B_7Series1/2
  Convert8/1 -> SOF_detector/1(ready)
  Assert1/1 -> Convert1/1  "Last"
  Mux1/1 -> GenericHighSpeedComm_Aurora_8B10B_7Series/1, fifo_tvalid/1
  Mux2/1 -> fifo_tdata/1, GenericHighSpeedComm_Aurora_8B10B_7Series/2
  Rate transition1/2 -> Mux1/2
  Rate transition1/1 -> Mux2/2
  Register1/1 -> Mux2/3
  SOF_detector/1(startofframe) -> Rate transition/5
  Constant8/1 -> Mux1/3
  Delay1/1 -> fifo_Trig/1, Rate transition1/5
  Delay3/1 -> GenericHighSpeedComm_Aurora_8B10B_7Series/3, fifo_tlast/1, Mux2/1, Mux1/1
  TimeStepSwitch/1(TimeStep) -> userTStep/1, Synchronization/1(Sync)
  TimestepGenerator/1(TimeStep) -> TimeStepSwitch/2(InitTimeStep)
  SofToAxi/1(Data) -> input_tdata/1, Rate transition1/1
  SofToAxi/2(Valid) -> "input_tvalid "/1, Rate transition1/2
  SofToAxi/3(Last) -> input_tlast/1, Rate transition1/3
  DataIN1/1 -> SofToAxi/1(DataIn)
  DataIN1/2 -> SofToAxi/2(SofIn)
